simulink model "AmpelkreuzungV5_99"  (R2024b)
settings: Solver=FixedStepAuto  StartTime=0.0  StopTime=5000  FixedStep=1  RelTol=1e-3
model workspace (MATLAB code in the model file):
  | function [autos_l1, autos_rg1, autos_2l, autos_2rg, autos_3l, autos_3rg, autos_4, fehler] = generateCars(Auslastung)
  |     if (auslastung == 1)
  |         autos_l1 = round(randn());
  |         autos_rg1 = round(randn());
  |         autos_2l = round(randn());
  |         autos_2rg = round(randn());
  |         autos_3l = round(randn());
  |         autos_3rg = round(randn());
  |         autos_4 = round(randn());
  |     else
  |         fehler = 1;
  |     end
  | 
  |     if (auslastung == 2)
  |         autos_l1 = round(randn());
  |         autos_rg1 = round(4 + 2 * randn());
  |         autos_2l = round(1 + randn());
  |         autos_2rg = round(4 + 2 * randn());
  |         autos_3l = round(randn());
  |         autos_3rg = round(2 + randn());
  |         autos_4 = round(1 + randn());
  |     else
  |         fehler = 1;
  |     end
  | 
  |     if (auslastung == 3)
  |         autos_l1 = round(1.5 + randn());
  |         autos_rg1 = round(7 + 2 * randn());
  |         autos_2l = round(2 + randn());
  |         autos_2rg = round(7 + 2 * randn());
  |         autos_3l = round(2 * randn());
  |         autos_3rg = round(3 + randn());
  |         autos_4 = round(2 + randn());
  |     else
  |         fehler = 1;
  |     end
  | 
  |     if (auslastung == 4)
  |         autos_l1 = round(2.5 + randn());
  |         autos_rg1 = round(13 + 3 * randn());
  |         autos_2l = round(5 + randn());
  |         autos_2rg = round(13 + 3 * randn());
  |         autos_3l = round(2 + randn());
  |         autos_3rg = round(2 + randn());
  |         autos_4 = round(5 + randn());
  |     else
  |         fehler = 1;
  |     end
  | end
(part 2 of 3)

== stateflow chart AmpelkreuzungV5_99/Chart ==
  state Start
    entry:
    clear all;
    rot1_l = 1;
    gelb1_l = 0;
    gruen1_l = 0;
    rot1_rg = 1;
    gelb1_rg = 0;
    gruen1_rg = 0;
    rot2 = 1;
    gelb2 = 0;
    gruen2 = 0;
    rot3_l = 1;
    gelb3_l = 0;
    gruen3_l = 0;
    rot3_rg = 1;
    gelb3_rg = 0;
    gruen3_rg = 0;
    rot4 = 1;
    gelb4 = 0;
    gruen4 = 0;
    rot5 = 1;
    gruen5 = 0;
    rot6 = 1;
    gruen6 = 0;
    rot7 = 1;
    gruen7 = 0;
    rot8 = 1;
    gruen8 = 0;
    timeCounter = 0;
    timer_spuren = [0 0 0 0 0 0 0];
    gesamtZeit = 0;
    gesamte_autos = 0;
    %alle_autos = [0 0 0 0 0 0 0; 0 0 0 0 0 0 0];
    spur1 = zeros(1,N / 2);
    spur2 = zeros(1,N / 2);
    spur3 = zeros(1,N / 2);
    spur4 = zeros(1,N / 2);
    spur5 = zeros(1,N / 2);
    spur6 = zeros(1,N / 2);
    spur7 = zeros(1,N / 2);
    autos_auf_spur1 = 0;
    autos_auf_spur2 = 0;
    autos_auf_spur3 = 0;
    autos_auf_spur4 = 0;
    autos_auf_spur5 = 0;
    autos_auf_spur6 = 0;
    autos_auf_spur7 = 0;
    counter = [0 0 0 0 0 0 0];
    anz_autos1 = 0;
    anz_autos2 = 0;
    anz_autos3 = 0;
    anz_autos4 = 0;
    anz_autos5 = 0;
    anz_autos6 = 0;
    anz_autos7 = 0;
    wartezeit_spur1_ges = 0;
    wartezeit_spur2_ges = 0;
    wartezeit_spur3_ges = 0;
    wartezeit_spur4_ges = 0;
    wartezeit_spur5_ges = 0;
    wartezeit_spur6_ges = 0;
    wartezeit_spur7_ges = 0;
    krit1 = 0;
    krit2 = 0;
    krit3 = 0;
  state dokumentiere_startzeiten_initialisiere_wartezeiten
    en:
    startzeiten1 = spur1;
    startzeiten2 = spur2;
    startzeiten3 = spur3;
    startzeiten4 = spur4;
    startzeiten5 = spur5;
    startzeiten6 = spur6;
    startzeiten7 = spur7;
    wartezeiten1 = zeros(1, length(startzeiten1));
    wartezeiten2 = zeros(1, length(startzeiten2));
    wartezeiten3 = zeros(1, length(startzeiten3));
    wartezeiten4 = zeros(1, length(startzeiten4));
    wartezeiten5 = zeros(1, length(startzeiten5));
    wartezeiten6 = zeros(1, length(startzeiten6));
    wartezeiten7 = zeros(1, length(startzeiten7));
  state endzeiten_initialisieren
    en:
    endzeiten1 = zeros(1, length(spur1));
    endzeiten2 = zeros(1, length(spur2));
    endzeiten3 = zeros(1, length(spur3));
    endzeiten4 = zeros(1, length(spur4));
    endzeiten5 = zeros(1, length(spur5));
    endzeiten6 = zeros(1, length(spur6));
    endzeiten7 = zeros(1, length(spur7));
  state rg1_ampel2_rotgelb
    entry:
    gelb1_rg = 1;
    gelb2 = 1;
  state l1_rg1_rotgelb
    entry:
    gelb1_l = 1;
    gelb1_rg = 1;
  state rg1_ampel2_gruen
    entry:
    rot1_rg = 0;
    gelb1_rg = 0;
    gruen1_rg = 1;
    rot2 = 0;
    gelb2 = 0;
    gruen2 = 1;
    rot7 = 0;
    gruen7 = 1;
    rot8 = 0;
    gruen8 = 1;
  state rg1_ampel2_rotgelb4
    entry:
    gelb1_rg = 1;
    gelb2 = 1;
  state l1_rg1_gruen
    entry:
    rot1_l = 0;
    gelb1_l = 0;
    gruen1_l = 1;
    rot1_rg = 0;
    gelb1_rg = 0;
    gruen1_rg = 1;
    rot7 = 0;
    gruen7 = 1;
  state l1_rg1_rotgelb4
    entry:
    gelb1_l = 1;
    gelb1_rg = 1;
  state rg1_ampel2_rotgelb1
    entry:
    gelb1_rg = 1;
    gelb2 = 1;
  state rg1_ampel2_gruen4
    entry:
    rot1_rg = 0;
    gelb1_rg = 0;
    gruen1_rg = 1;
    rot2 = 0;
    gelb2 = 0;
    gruen2 = 1;
    rot7 = 0;
    gruen7 = 1;
    rot8 = 0;
    gruen8 = 1;
  state l1_rg1_rotgelb1
    entry:
    gelb1_l = 1;
    gelb1_rg = 1;
  state l1_gelb
    entry:
    gelb1_l = 1;
    gruen1_l = 0;
  state rg1_ampel2_gruen1
    entry:
    rot1_rg = 0;
    gelb1_rg = 0;
    gruen1_rg = 1;
    rot2 = 0;
    gelb2 = 0;
    gruen2 = 1;
    rot7 = 0;
    gruen7 = 1;
    rot8 = 0;
    gruen8 = 1;
  state l1_rg1_gruen4
    entry:
    rot1_l = 0;
    gelb1_l = 0;
    gruen1_l = 1;
    rot1_rg = 0;
    gelb1_rg = 0;
    gruen1_rg = 1;
    rot7 = 0;
    gruen7 = 1;
  state l1_rg1_gruen1
    entry:
    rot1_l = 0;
    gelb1_l = 0;
    gruen1_l = 1;
    rot1_rg = 0;
    gelb1_rg = 0;
    gruen1_rg = 1;
    rot7 = 0;
    gruen7 = 1;
  state rg1_ampel2_rotgelb3
    entry:
    gelb1_rg = 1;
    gelb2 = 1;
  state l1_rot
    entry:
    rot1_l = 1;
    gelb1_l = 0;
  state l1_rg1_rotgelb3
    entry:
    gelb1_l = 1;
    gelb1_rg = 1;
  state Fuss7_rot1
    entry:
    rot7 = 1;
    gruen7 = 0;
  state l1_gelb4
    entry:
    gelb1_l = 1;
    gruen1_l = 0;
  state rg1_ampel2_gruen3
    entry:
    rot1_rg = 0;
    gelb1_rg = 0;
    gruen1_rg = 1;
    rot2 = 0;
    gelb2 = 0;
    gruen2 = 1;
    rot7 = 0;
    gruen7 = 1;
    rot8 = 0;
    gruen8 = 1;
  state l1_gelb1
    entry:
    gelb1_l = 1;
    gruen1_l = 0;
  state l1_rg1_gruen3
    entry:
    rot1_l = 0;
    gelb1_l = 0;
    gruen1_l = 1;
    rot1_rg = 0;
    gelb1_rg = 0;
    gruen1_rg = 1;
    rot7 = 0;
    gruen7 = 1;
  state l1_rot1
    entry:
    rot1_l = 1;
    gelb1_l = 0;
  state l1_rot9
    entry:
    rot1_l = 1;
    gelb1_l = 0;
  state rg1_gelb1
    entry:
    gelb1_rg = 1;
    gruen1_rg = 0;
  state Fuss7_rot8
    entry:
    rot7 = 1;
    gruen7 = 0;
  state l1_rot2
    entry:
    rot1_l = 1;
    gelb1_l = 0;
  state ampel2_rotgelb
    entry:
    gelb2 = 1;
  state Fuss7_rot2
    entry:
    rot7 = 1;
    gruen7 = 0;
  state ampel2_fuss8_gruen
    rot2 = 0;
    gelb2 = 0;
    gruen2 = 1;
    rot8 = 0;
    gruen8 = 1;
  state l1_gelb3
    entry:
    gelb1_l = 1;
    gruen1_l = 0;
  state rg1_rot1
    entry:
    gelb1_rg = 0;
    rot1_rg = 1;
  state l1_rot8
    entry:
    rot1_l = 1;
    gelb1_l = 0;
  state rg1_gelb9
    entry:
    gelb1_rg = 1;
    gruen1_rg = 0;
  state l1_rot3
    entry:
    rot1_l = 1;
    gelb1_l = 0;
  state ampel2_rotgelb4
    entry:
    gelb2 = 1;
  state rg1_gelb2
    entry:
    gelb1_rg = 1;
    gruen1_rg = 0;
  state l1_rot6
    entry:
    rot1_l = 1;
    gelb1_l = 0;
  state Fuss7_rot6
    entry:
    rot7 = 1;
    gruen7 = 0;
  state ampel2_rotgelb1
    entry:
    gelb2 = 1;
  state ampel2_fuss8_gruen4
    rot2 = 0;
    gelb2 = 0;
    gruen2 = 1;
    rot8 = 0;
    gruen8 = 1;
  state rg1_rot23
    entry:
    gelb1_rg = 0;
    rot1_rg = 1;
  state ampel2_fuss8_gruen1
    rot2 = 0;
    gelb2 = 0;
    gruen2 = 1;
    rot8 = 0;
    gruen8 = 1;
  state Fuss7_rot
    entry:
    rot7 = 1;
    gruen7 = 0;
  state rg1_rot6
    entry:
    gelb1_rg = 0;
    rot1_rg = 1;
  state l1_rot7
    entry:
    rot1_l = 1;
    gelb1_l = 0;
  state rg1_gelb7
    entry:
    gelb1_rg = 1;
    gruen1_rg = 0;
  state rg1_gelb
    entry:
    gelb1_rg = 1;
    gruen1_rg = 0;
  state fuss7_rot
    entry:
    rot7 = 1;
    gruen7 = 0;
  state Fuss7_rot7
    entry:
    rot7 = 1;
    gruen7 = 0;
  state rg1_rot20
    entry:
    gelb1_rg = 0;
    rot1_rg = 1;
  state rg1_rot
    entry:
    gelb1_rg = 0;
    rot1_rg = 1;
  state Fuss7_rot3
    entry:
    rot7 = 1;
    gruen7 = 0;
  state rg1_rot5
    entry:
    gelb1_rg = 0;
    rot1_rg = 1;
  state rg1_gelb8
    entry:
    gelb1_rg = 1;
    gruen1_rg = 0;
  state ampel2_rotgelb3
    entry:
    gelb2 = 1;
  state rg1_gelb3
    entry:
    gelb1_rg = 1;
    gruen1_rg = 0;
  state ampel2_fuss8_gruen3
    rot2 = 0;
    gelb2 = 0;
    gruen2 = 1;
    rot8 = 0;
    gruen8 = 1;
  state rg1_rot26
    entry:
    gelb1_rg = 0;
    rot1_rg = 1;
  state rg1_rot7
    entry:
    gelb1_rg = 0;
    rot1_rg = 1;
  state fuss8_rot7
    entry:
    rot8 = 1;
    gruen8 = 0;
  state rg1_rot4
    entry:
    gelb1_rg = 0;
    rot1_rg = 1;
  state rg1_gelb6
    entry:
    gelb1_rg = 1;
    gruen1_rg = 0;
  state rg1_rot11
    entry:
    gelb1_rg = 0;
    rot1_rg = 1;
  state rg1_rot17
    entry:
    gelb1_rg = 0;
    rot1_rg = 1;
  state rg1_rot22
    entry:
    gelb1_rg = 0;
    rot1_rg = 1;
  state fuss8_rot11
    entry:
    rot8 = 1;
    gruen8 = 0;
  state rg1_rot9
    entry:
    gelb1_rg = 0;
    rot1_rg = 1;
  state fuss8_rot13
    entry:
    rot8 = 1;
    gruen8 = 0;
  state rg1_rot24
    entry:
    gelb1_rg = 0;
    rot1_rg = 1
  state fuss8_rot14
    entry:
    rot8 = 1;
    gruen8 = 0;
  state rg1_rot25
    entry:
    gelb1_rg = 0;
    rot1_rg = 1
  state rg1_rot21
    entry:
    gelb1_rg = 0;
    rot1_rg = 1;
  state fuss8_rot5
    entry:
    rot8 = 1;
    gruen8 = 0;
  state fuss8_rot4
    entry:
    rot8 = 1;
    gruen8 = 0;
  state ampel2_gelb12
    entry:
    gelb2 = 1;
    gruen2 = 0;
  state ampel2_gelb13
    entry:
    gelb2 = 1;
    gruen2 = 0;
  state ampel2_gelb5
    entry:
    gelb2 = 1;
    gruen2 = 0;
  state ampel2_gelb4
    entry:
    gelb2 = 1;
    gruen2 = 0;
  state rg1_rot19
    entry:
    gelb1_rg = 0;
    rot1_rg = 1
  state ampel2_gelb8
    entry:
    gelb2 = 1;
    gruen2 = 0;
  state rg1_rot3
    entry:
    gelb1_rg = 0;
    rot1_rg = 1
  state rg1_rot18
    entry:
    gelb1_rg = 0;
    rot1_rg = 1
  state ampel2_gelb11
    entry:
    gelb2 = 1;
    gruen2 = 0;
  state rg1_rot2
    entry:
    gelb1_rg = 0;
    rot1_rg = 1
  state fuss8_rot10
    entry:
    rot8 = 1;
    gruen8 = 0;
  state fuss8_rot12
    entry:
    rot8 = 1;
    gruen8 = 0;
  state ampel2_rot24
    rot2 = 1;
    gelb2 = 0;
  state fuss8_rot1
    entry:
    rot8 = 1;
    gruen8 = 0;
  state ampel2_rot11
    rot2 = 1;
    gelb2 = 0;
  state fuss8_rot
    entry:
    rot8 = 1;
    gruen8 = 0;
  state ampel2_gelb9
    entry:
    gelb2 = 1;
    gruen2 = 0;
  state ampel2_gelb10
    entry:
    gelb2 = 1;
    gruen2 = 0;
  state ampel2_gelb1
    entry:
    gelb2 = 1;
    gruen2 = 0;
  state rg1_rot8
    entry:
    gelb1_rg = 0;
    rot1_rg = 1
  state ampel2_gelb
    entry:
    gelb2 = 1;
    gruen2 = 0;
  state rg1_rot10
    entry:
    gelb1_rg = 0;
    rot1_rg = 1
  state ampel2_rot25
    rot2 = 1;
    gelb2 = 0;
  state ampel2_rot9
    rot2 = 1;
    gelb2 = 0;
  state fuss8_rot3
    entry:
    rot8 = 1;
    gruen8 = 0;
  state ampel2_rot19
    rot2 = 1;
    gelb2 = 0;
  state fuss8_rot2
    entry:
    rot8 = 1;
    gruen8 = 0;
  state ampel2_rot17
    rot2 = 1;
    gelb2 = 0;
  state ampel2_rot
    rot2 = 1;
    gelb2 = 0;
  state ampel2_gelb3
    entry:
    gelb2 = 1;
    gruen2 = 0;
  state ampel2_gelb2
    entry:
    gelb2 = 1;
    gruen2 = 0;
  state ampel2_rot21
    rot2 = 1;
    gelb2 = 0;
  state ampel2_rot20
    rot2 = 1;
    gelb2 = 0;
  state ampel2_rot1
    rot2 = 1;
    gelb2 = 0;
  state ampel2_rot5
    rot2 = 1;
    gelb2 = 0;
  state ampel2_rot26
    rot2 = 1;
    gelb2 = 0;
  state ampel2_rot10
    rot2 = 1;
    gelb2 = 0;
  state ampel2_rot27
    rot2 = 1;
    gelb2 = 0;
  state ampel2_rot8
    rot2 = 1;
    gelb2 = 0;
  state rg3_rotgelb13
    entry:
    gelb3_rg = 1;
  state rg3_rotgelb4
    entry:
    gelb3_rg = 1;
  state ampel2_rot6
    rot2 = 1;
    gelb2 = 0;
  state rg3_rotgelb14
    entry:
    gelb3_rg = 1;
  state rg3_rotgelb5
    entry:
    gelb3_rg = 1;
  state ampel2_rot16
    rot2 = 1;
    gelb2 = 0;
  state ampel2_rot22
    rot2 = 1;
    gelb2 = 0;
  state ampel2_rot18
    rot2 = 1;
    gelb2 = 0;
  state ampel2_rot2
    rot2 = 1;
    gelb2 = 0;
  state ampel2_rot23
    rot2 = 1;
    gelb2 = 0;
  state ampel2_rot3
    rot2 = 1;
    gelb2 = 0;
  state rg3_rotgelb10
    entry:
    gelb3_rg = 1;
  state rg3_rotgelb11
    entry:
    gelb3_rg = 1;
  state rg3_rotgelb12
    entry:
    gelb3_rg = 1;
  state rg3_rotgelb
    entry:
    gelb3_rg = 1;
  state rg3_rotgelb9
    entry:
    gelb3_rg = 1;
  state rg3_rotgelb1
    entry:
    gelb3_rg = 1;
  state ampel2_rot7
    rot2 = 1;
    gelb2 = 0;
  state ampel2_rot4
    rot2 = 1;
    gelb2 = 0;
  state rg3_rotgelb2
    entry:
    gelb3_rg = 1;
  state l3_rotgelb_rg3_fuss6_gruen
    entry:
    gelb3_l = 1;
    rot3_rg = 0;
    gelb3_rg = 0;
    gruen3_rg = 1;
    rot6 = 0;
    gruen6 = 1;
  state rg3_fuss6_gruen
    entry:
    rot3_rg = 0;
    gelb3_rg = 0;
    gruen3_rg = 1;
    rot6 = 0;
    gruen6 = 1;
  state rg3_rotgelb3
    entry:
    gelb3_rg = 1;
  state rg3_rotgelb6
    entry:
    gelb3_rg = 1;
  state ampel4_rotgelb
    entry:
    gelb4 = 1;
  state l3_rotgelb_rg3_fuss6_gruen4
    entry:
    gelb3_l = 1;
    rot3_rg = 0;
    gelb3_rg = 0;
    gruen3_rg = 1;
    rot6 = 0;
    gruen6 = 1;
  state rg3_fuss6_gruen4
    entry:
    rot3_rg = 0;
    gelb3_rg = 0;
    gruen3_rg = 1;
    rot6 = 0;
    gruen6 = 1;
  state l3_gruen
    entry:
    rot3_l = 0;
    gelb3_l = 0;
    gruen3_l = 1;
  state l3_rotgelb_rg3_fuss6_gruen1
    entry:
    gelb3_l = 1;
    rot3_rg = 0;
    gelb3_rg = 0;
    gruen3_rg = 1;
    rot6 = 0;
    gruen6 = 1;
  state rg3_fuss6_gruen1
    entry:
    rot3_rg = 0;
    gelb3_rg = 0;
    gruen3_rg = 1;
    rot6 = 0;
    gruen6 = 1;
  state ampel4_rotgelb4
    entry:
    gelb4 = 1;
  state l3_gruen4
    entry:
    rot3_l = 0;
    gelb3_l = 0;
    gruen3_l = 1;
  state l3_gelb
    entry:
    gelb3_l = 1;
    gruen3_l = 0;
  state ampel4_rotgelb1
    entry:
    gelb4 = 1;
  state l3_gruen1
    entry:
    rot3_l = 0;
    gelb3_l = 0;
    gruen3_l = 1;
  state ampel4_fuss5_gruen
    entry:
    rot4 = 0;
    gelb4 = 0;
    gruen4 = 1;
    rot5 = 0;
    gruen5 = 1;
  state l3_rotgelb_rg3_fuss6_gruen3
    entry:
    gelb3_l = 1;
    rot3_rg = 0;
    gelb3_rg = 0;
    gruen3_rg = 1;
    rot6 = 0;
    gruen6 = 1;
  state rg3_fuss6_gruen3
    entry:
    rot3_rg = 0;
    gelb3_rg = 0;
    gruen3_rg = 1;
    rot6 = 0;
    gruen6 = 1;
  state l3_fuss6_rot
    entry:
    rot3_l = 1;
    gelb3_l = 0;
    rot6 = 1;
    gruen6 = 0;
  state l3_gelb_fuss6_rot
    entry:
    gelb3_l = 1;
    gruen3_l = 0;
  state ampel4_rotgelb3
    entry:
    gelb4 = 1;
  state ampel4_fuss5_gruen8
    entry:
    rot4 = 0;
    gelb4 = 0;
    gruen4 = 1;
    rot5 = 0;
    gruen5 = 1;
  state l3_gelb1
    entry:
    gelb3_l = 1;
    gruen3_l = 0;
  state l3_gruen3
    entry:
    rot3_l = 0;
    gelb3_l = 0;
    gruen3_l = 1;
  state fuss6_rot6
    entry:
    rot6 = 1;
    gruen6 = 0;
  state ampel4_fuss5_gruen2
    entry:
    rot4 = 0;
    gelb4 = 0;
    gruen4 = 1;
    rot5 = 0;
    gruen5 = 1;
  state l3_fuss6_rot3
    entry:
    rot3_l = 1;
    gelb3_l = 0;
    rot6 = 1;
    gruen6 = 0;
  state l3_rot1
    entry:
    rot3_l = 1;
    gelb3_l = 0;
  state l3_gelb2
    entry:
    gelb3_l = 1;
    gruen3_l = 0;
  state l3_fuss6_rot1
    entry:
    rot3_l = 1;
    gelb3_l = 0;
    rot6 = 1;
    gruen6 = 0;
  state ampel4_fuss5_gruen6
    entry:
    rot4 = 0;
    gelb4 = 0;
    gruen4 = 1;
    rot5 = 0;
    gruen5 = 1;
  state fuss6_rot
    entry:
    rot6 = 1;
    gruen6 = 0;
  state fuss6_rot4
    entry:
    rot6 = 1;
    gruen6 = 0;
  state rg3_gelb1
    entry:
    gelb3_rg = 1;
    gruen3_rg = 0;
  state rg3_gelb
    entry:
    gelb3_rg = 1;
    gruen3_rg = 0;
  state l3_rot_rg3_gelb
    entry:
    rot3_l = 1;
    gelb3_l = 0;
    gelb3_rg = 1;
    gruen3_rg = 0;
  state l3_rot
    entry:
    rot3_l = 1;
    gelb3_l = 0;
  state fuss6_rot7
    entry:
    rot6 = 1;
    gruen6 = 0;
  state l3_fuss6_rot2
    entry:
    rot3_l = 1;
    gelb3_l = 0;
    rot6 = 1;
    gruen6 = 0;
  state fuss6_rot1
    entry:
    rot6 = 1;
    gruen6 = 0;
  state rg3_gelb8
    entry:
    gelb3_rg = 1;
    gruen3_rg = 0;
  state rg3_gelb7
    entry:
    gelb3_rg = 1;
    gruen3_rg = 0;
  state rg3_rot_ampel4_rotgelb
    entry:
    rot3_rg = 1;
    gelb3_rg = 0;
    gelb4 = 1;
  state rg3_gelb2
    entry:
    gelb3_rg = 1;
    gruen3_rg = 0;
  state rg3_gelb3
    entry:
    gelb3_rg = 1;
    gruen3_rg = 0;
  state rg3_fuss5_rot
    entry:
    rot3_rg = 1;
    gelb3_rg = 0;
    rot5 = 1;
    gruen5 = 0;
  state fuss6_rot5
    entry:
    rot6 = 1;
    gruen6 = 0;
  state rg3_rot_ampel4_rotgelb8
    entry:
    rot3_rg = 1;
    gelb3_rg = 0;
    gelb4 = 1;
  state l3_rot_rg3_gelb1
    entry:
    rot3_l = 1;
    gelb3_l = 0;
    gelb3_rg = 1;
    gruen3_rg = 0;
  state rg3_gelb6
    entry:
    gelb3_rg = 1;
    gruen3_rg = 0;
  state rg3_rot_ampel4_rotgelb2
    entry:
    rot3_rg = 1;
    gelb3_rg = 0;
    gelb4 = 1;
  state rg3_fuss5_rot8
    entry:
    rot3_rg = 1;
    gelb3_rg = 0;
    rot5 = 1;
    gruen5 = 0;
  state rg3_rot_ampel4_rotgelb1
    entry:
    rot3_rg = 1;
    gelb3_rg = 0;
    gelb4 = 1;
  state rg3_fuss5_rot2
    entry:
    rot3_rg = 1;
    gelb3_rg = 0;
    rot5 = 1;
    gruen5 = 0;
  state rg3_rot_ampel4_rotgelb6
    entry:
    rot3_rg = 1;
    gelb3_rg = 0;
    gelb4 = 1;
  state ampel4_fuss5_gruen1
    entry:
    rot4 = 0;
    gelb4 = 0;
    gruen4 = 1;
    rot5 = 0;
    gruen5 = 1;
  state rg3_rot_ampel4_rotgelb9
    entry:
    rot3_rg = 1;
    gelb3_rg = 0;
    gelb4 = 1;
  state rg3_fuss5_rot6
    entry:
    rot3_rg = 1;
    gelb3_rg = 0;
    rot5 = 1;
    gruen5 = 0;
  state rg3_rot_ampel4_rotgelb3
    entry:
    rot3_rg = 1;
    gelb3_rg = 0;
    gelb4 = 1;
  state ampel4_fuss5_gruen9
    entry:
    rot4 = 0;
    gelb4 = 0;
    gruen4 = 1;
    rot5 = 0;
    gruen5 = 1;
  state fuss5_rot
    entry:
    rot5 = 1;
    gruen5 = 0;
  state ampel4_fuss5_gruen3
    entry:
    rot4 = 0;
    gelb4 = 0;
    gruen4 = 1;
    rot5 = 0;
    gruen5 = 1;
  state rg3_rot_ampel4_rotgelb7
    entry:
    rot3_rg = 1;
    gelb3_rg = 0;
    gelb4 = 1;
  state rg3_fuss5_rot1
    entry:
    rot3_rg = 1;
    gelb3_rg = 0;
    rot5 = 1;
    gruen5 = 0;
  state fuss5_rot4
    entry:
    rot5 = 1;
    gruen5 = 0;
  state ampel4_fuss5_gruen7
    entry:
    rot4 = 0;
    gelb4 = 0;
    gruen4 = 1;
    rot5 = 0;
    gruen5 = 1;
  state fuss5_rot1
    entry:
    rot5 = 1;
    gruen5 = 0;
  state rg3_fuss5_rot9
    entry:
    rot3_rg = 1;
    gelb3_rg = 0;
    rot5 = 1;
    gruen5 = 0;
  state rg3_fuss5_rot3
    entry:
    rot3_rg = 1;
    gelb3_rg = 0;
    rot5 = 1;
    gruen5 = 0;
  state fuss5_rot3
    entry:
    rot5 = 1;
    gruen5 = 0;
  state ampel4_gelb
    entry:
    gelb4 = 1;
    gruen4 = 0;
  state rg3_fuss5_rot7
    entry:
    rot3_rg = 1;
    gelb3_rg = 0;
    rot5 = 1;
    gruen5 = 0;
  state ampel4_rot
    entry:
    rot4 = 1;
    gelb4 = 0;
  state ampel4_gelb4
    entry:
    gelb4 = 1;
    gruen4 = 0;
  state ampel4_rot2
    entry:
    rot4 = 1;
    gelb4 = 0;
  state ampel4_gelb1
    entry:
    gelb4 = 1;
    gruen4 = 0;
  state ampel4_rot9
    entry:
    rot4 = 1;
    gelb4 = 0;
  state ampel4_rot3
    entry:
    rot4 = 1;
    gelb4 = 0;
  state ampel4_rot10
    entry:
    rot4 = 1;
    gelb4 = 0;
  state ampel4_gelb3
    entry:
    gelb4 = 1;
    gruen4 = 0;
  state ampel4_rot4
    entry:
    rot4 = 1;
    gelb4 = 0;
  state ampel4_rot7
    entry:
    rot4 = 1;
    gelb4 = 0;
  state ampel4_rot8
    entry:
    rot4 = 1;
    gelb4 = 0;
  (default) -> Start
  Start -> (junction 796) : {zeit_abstand = zeit_abstand_aus_auslastung(auslastung);}
  (junction 796) -> (junction 748) : {alle_autos_neu  = generiere_autos_neu(N, zeit_abstand, auslastung);}
  (junction 748) -> dokumentiere_startzeiten_initialisiere_wartezeiten : {[spur1, spur2, spur3, spur4, spur5, spur6, spur7] = spuren_aus_autos(alle_autos_neu, N);}
  dokumentiere_startzeiten_initialisiere_wartezeiten -> endzeiten_initialisieren
  endzeiten_initialisieren -> (junction 248)
  (junction 181) -> (junction 248) : {timeCounter = resetTimer()}
  (junction 248) -> (junction 1426) [order 1] : [auslastung == 5]
  (junction 248) -> (junction 1428) [order 2]
  (junction 179) -> (junction 181)
  (junction 1426) -> (junction 1092) : {alte_counter = counter;}
  (junction 1428) -> (junction 1430) [order 1] : [auslastung == 4]
  (junction 1428) -> (junction 1840) [order 2]
  (junction 1430) -> (junction 1670) : {alte_counter = counter;}
  (junction 1840) -> (junction 1843) [order 1] : [auslastung == 3]
  (junction 1840) -> (junction 3331) [order 2]
  (junction 1843) -> (junction 3396) : {alte_counter = counter;}
  (junction 3331) -> (junction 3333) : [auslastung == 1 || auslastung == 2]
  (junction 3333) -> (junction 3239) : {alte_counter = counter;}
  (junction 1092) -> (junction 1075) : after(1,sec)
      | {timeCounter = refresher(timeCounter, 1);}
  (junction 1075) -> (junction 1077) : {timer_spuren = countOnwards(timer_spuren,1,[1 1 1 1 1 1 1]);}
      |
      | %Linksabbieger1
  (junction 1077) -> (junction 1076) : {[autos_auf_spur1, spur1] = autos_auf_spur_generieren(spur1, gesamtZeit + timeCounter + 2, autos_auf_spur1);}
  (junction 3396) -> (junction 3418) : after(1,sec)
      | {timeCounter = refresher(timeCounter, 1);}
  (junction 1076) -> (junction 1081) : {autos_spur1_flag = false;}
  (junction 3418) -> (junction 3423) : {timer_spuren = countOnwards(timer_spuren,1,[1 1 1 1 1 1 1]);}
      |
      | %Linksabbieger1
  (junction 1670) -> (junction 1696) : after(1,sec)
      | {timeCounter = refresher(timeCounter, 1);}
  (junction 1081) -> (junction 1085) [order 1] : [autos_auf_spur1 == 0]
  (junction 1696) -> (junction 1673) : {timer_spuren = countOnwards(timer_spuren,1,[1 1 1 1 1 1 1]);}
      |
      | %Linksabbieger1
  (junction 3423) -> (junction 3398) : {[autos_auf_spur1, spur1] = autos_auf_spur_generieren(spur1, gesamtZeit + timeCounter + 2, autos_auf_spur1);}
  (junction 1081) -> (junction 1084) [order 2]
  (junction 1085) -> rg1_ampel2_rotgelb
  (junction 1084) -> (junction 1074) [order 1] : [autos_auf_spur1 > 0]
  (junction 1084) -> (junction 1111) [order 2]
  (junction 1074) -> l1_rg1_rotgelb : {autos_spur1_flag = true;}
  rg1_ampel2_rotgelb -> (junction 1097) : after(1,sec)
      | {timeCounter = refresher(timeCounter, 1);}
  (junction 1673) -> (junction 1668) : {[autos_auf_spur1, spur1] = autos_auf_spur_generieren(spur1, gesamtZeit + timeCounter + 2, autos_auf_spur1);}
  (junction 1097) -> rg1_ampel2_gruen : {timer_spuren = countOnwards(timer_spuren,1,[1 1 1 1 1 1 1]);}
  (junction 3398) -> (junction 3386) : {autos_spur1_flag = false;}
  l1_rg1_rotgelb -> (junction 1082) : after(1,sec)
      | {timeCounter = refresher(timeCounter, 1);}
  (junction 1082) -> l1_rg1_gruen : {timer_spuren = countOnwards(timer_spuren,1,[1 1 1 1 1 1 1]);}
  (junction 3239) -> (junction 3238) : after(1,sec)
      | {timeCounter = refresher(timeCounter, 1);}
  (junction 1668) -> (junction 1687) : {autos_spur1_flag = false;}
  (junction 3386) -> (junction 3402) [order 1] : [autos_auf_spur1 == 0]
  (junction 3402) -> rg1_ampel2_rotgelb4
  (junction 3386) -> (junction 3387) [order 2]
  (junction 3238) -> (junction 3241) : {timer_spuren = countOnwards(timer_spuren,1,[1 1 1 1 1 1 1]);}
      |
      | %Linksabbieger1
  (junction 3387) -> (junction 3395) [order 1] : [autos_auf_spur1 > 0]
  (junction 3387) -> (junction 3436) [order 2]
  (junction 3395) -> l1_rg1_rotgelb4 : {autos_spur1_flag = true;}
  rg1_ampel2_rotgelb4 -> (junction 3400) : after(1,sec)
      | {timeCounter = refresher(timeCounter, 1);}
  rg1_ampel2_gruen -> (junction 1080) : {[autos_auf_spur2, spur2] = autos_auf_spur_generieren(spur2, gesamtZeit + timeCounter, autos_auf_spur2);}
  (junction 1687) -> (junction 1688) [order 1] : [autos_auf_spur1 == 0]
  (junction 1687) -> (junction 1690) [order 2]
  (junction 1688) -> rg1_ampel2_rotgelb1
  (junction 3241) -> (junction 3240) : {[autos_auf_spur1, spur1] = autos_auf_spur_generieren(spur1, gesamtZeit + timeCounter + 2, autos_auf_spur1);}
  (junction 1080) -> (junction 1098) : {[autos_auf_spur3, spur3] = autos_auf_spur_generieren(spur3, gesamtZeit + timeCounter, autos_auf_spur3);}
  (junction 3400) -> rg1_ampel2_gruen4 : {timer_spuren = countOnwards(timer_spuren,1,[1 1 1 1 1 1 1]);}
  l1_rg1_gruen -> (junction 1083) : {[autos_auf_spur1, spur1] = autos_auf_spur_generieren(spur1, gesamtZeit + timeCounter, autos_auf_spur1);}
  (junction 1690) -> (junction 1697) [order 1] : [autos_auf_spur1 > 0]
  (junction 1690) -> (junction 1741) [order 2]
  (junction 1697) -> l1_rg1_rotgelb1 : {autos_spur1_flag = true;}
  l1_rg1_rotgelb4 -> (junction 3404) : after(1,sec)
      | {timeCounter = refresher(timeCounter, 1);}
  rg1_ampel2_rotgelb1 -> (junction 1698) : after(1,sec)
      | {timeCounter = refresher(timeCounter, 1);}
  (junction 1083) -> (junction 1078) : {[autos_auf_spur2, spur2] = autos_auf_spur_generieren(spur2, gesamtZeit + timeCounter, autos_auf_spur2);}
  (junction 1098) -> (junction 1086) : {[autos_auf_spur4, spur4] = autos_auf_spur_generieren(spur4, gesamtZeit + timeCounter, autos_auf_spur4);}
  (junction 3404) -> l1_rg1_gruen4 : {timer_spuren = countOnwards(timer_spuren,1,[1 1 1 1 1 1 1]);}
  (junction 1078) -> (junction 1073) : after(8,sec)
      | {timeCounter = refresher(timeCounter, 8);}
  (junction 1698) -> rg1_ampel2_gruen1 : {timer_spuren = countOnwards(timer_spuren,1,[1 1 1 1 1 1 1]);}
  l1_rg1_rotgelb1 -> (junction 1715) : after(1,sec)
      | {timeCounter = refresher(timeCounter, 1);}
  (junction 3240) -> (junction 3243) : {autos_spur1_flag = false;}
  (junction 1073) -> l1_gelb : {timer_spuren = countOnwards(timer_spuren,8,[0 0 1 1 1 1 1]);}
  (junction 1086) -> (junction 1087) : after(45,sec)
      | {timeCounter = refresher(timeCounter, 45);}
  (junction 1715) -> l1_rg1_gruen1 : {timer_spuren = countOnwards(timer_spuren,1,[1 1 1 1 1 1 1]);}
  l1_gelb -> (junction 1093) : after(3,sec)
      | {timeCounter = refresher(timeCounter, 3);}
  (junction 1087) -> Fuss7_rot1 : {timer_spuren = countOnwards(timer_spuren,45,[1 0 0 0 1 1 1]);}
  rg1_ampel2_gruen4 -> (junction 3408) : {[autos_auf_spur2, spur2] = autos_auf_spur_generieren(spur2, gesamtZeit + timeCounter, autos_auf_spur2);}
  (junction 1093) -> (junction 1079) : {[autos_auf_spur1, spur1] = autos_auf_spur_generieren(spur1, gesamtZeit + timeCounter, autos_auf_spur1);}
  (junction 3243) -> (junction 3249) [order 1] : [autos_auf_spur1 == 0]
  (junction 3243) -> (junction 3244) [order 2]
  (junction 3249) -> rg1_ampel2_rotgelb3
  (junction 3408) -> (junction 3441) : {[autos_auf_spur3, spur3] = autos_auf_spur_generieren(spur3, gesamtZeit + timeCounter, autos_auf_spur3);}
  (junction 1079) -> l1_rot : {timer_spuren = countOnwards(timer_spuren,3,[0 0 1 1 1 1 1]);}
  l1_rg1_gruen4 -> (junction 3414) : {[autos_auf_spur1, spur1] = autos_auf_spur_generieren(spur1, gesamtZeit + timeCounter, autos_auf_spur1);}
  (junction 3244) -> (junction 3245) [order 1] : [autos_auf_spur1 > 0]
  rg1_ampel2_gruen1 -> (junction 1704) : {[autos_auf_spur2, spur2] = autos_auf_spur_generieren(spur2, gesamtZeit + timeCounter, autos_auf_spur2);}
  (junction 3244) -> (junction 3120) [order 2]
  (junction 3245) -> l1_rg1_rotgelb3 : {autos_spur1_flag = true;}
  rg1_ampel2_rotgelb3 -> (junction 3246) : after(1,sec)
      | {timeCounter = refresher(timeCounter, 1);}
  (junction 3414) -> (junction 3438) : {[autos_auf_spur2, spur2] = autos_auf_spur_generieren(spur2, gesamtZeit + timeCounter, autos_auf_spur2);}
  (junction 3441) -> (junction 3454) : {[autos_auf_spur4, spur4] = autos_auf_spur_generieren(spur4, gesamtZeit + timeCounter, autos_auf_spur4);}
  l1_rot -> (junction 1095) : {[anz_autos1, autos_auf_spur1, counter(1), endzeiten1] = generiere_gruenphase(1, 11, autos_auf_spur1, counter(1),  (gesamtZeit + timeCounter - 11), endzeiten1, startzeiten1, auslastung, autos_spur1_flag);}
  (junction 1704) -> (junction 1722) : {[autos_auf_spur3, spur3] = autos_auf_spur_generieren(spur3, gesamtZeit + timeCounter, autos_auf_spur3);}
  (junction 3438) -> (junction 3442) : after(8,sec)
      | {timeCounter = refresher(timeCounter, 8);}
  l1_rg1_gruen1 -> (junction 1720) : {[autos_auf_spur1, spur1] = autos_auf_spur_generieren(spur1, gesamtZeit + timeCounter, autos_auf_spur1);}
  (junction 3246) -> rg1_ampel2_gruen3 : {timer_spuren = countOnwards(timer_spuren,1,[1 1 1 1 1 1 1]);}
  (junction 1095) -> (junction 1096) : {wartezeiten1 = berechne_wartezeiten(startzeiten1, endzeiten1, alte_counter(1), counter(1), wartezeiten1);}
  (junction 3454) -> (junction 3426) : after(20,sec)
      | {timeCounter = refresher(timeCounter, 20);}
  l1_rg1_rotgelb3 -> (junction 3247) : after(1,sec)
      | {timeCounter = refresher(timeCounter, 1);}
  (junction 3442) -> l1_gelb4 : {timer_spuren = countOnwards(timer_spuren,8,[0 0 1 1 1 1 1]);}
  (junction 1720) -> (junction 1711) : {[autos_auf_spur2, spur2] = autos_auf_spur_generieren(spur2, gesamtZeit + timeCounter, autos_auf_spur2);}
  (junction 1722) -> (junction 1712) : {[autos_auf_spur4, spur4] = autos_auf_spur_generieren(spur4, gesamtZeit + timeCounter, autos_auf_spur4);}
  (junction 1096) -> (junction 1099) : {wartezeit_spur1_ges = gesamt_wartezeit_pro_spur(wartezeiten1, wartezeit_spur1_ges, alte_counter(1), counter(1));}
  Fuss7_rot1 -> (junction 1072) : after(2,sec)
      | {timeCounter = refresher(timeCounter, 2);}
  (junction 3247) -> l1_rg1_gruen3 : {timer_spuren = countOnwards(timer_spuren,1,[1 1 1 1 1 1 1]);}
  (junction 1711) -> (junction 1721) : after(8,sec)
      | {timeCounter = refresher(timeCounter, 8);}
  (junction 3426) -> Fuss7_rot8 : {timer_spuren = countOnwards(timer_spuren,20,[1 0 0 0 1 1 1]);}
  l1_gelb4 -> (junction 3439) : after(3,sec)
      | {timeCounter = refresher(timeCounter, 3);}
  (junction 1099) -> (junction 1090) : {gesamtwartezeit = berechne_gesamtwartezeit(wartezeit_spur1_ges, wartezeit_spur2_ges, wartezeit_spur3_ges, wartezeit_spur4_ges, wartezeit_spur5_ges, wartezeit_spur6_ges, wartezeit_spur7_ges);}
  (junction 1721) -> l1_gelb1 : {timer_spuren = countOnwards(timer_spuren,8,[0 0 1 1 1 1 1]);}
  (junction 1712) -> (junction 1723) : after(35,sec)
      | {timeCounter = refresher(timeCounter, 35);}
  (junction 3439) -> (junction 3452) : {[autos_auf_spur1, spur1] = autos_auf_spur_generieren(spur1, gesamtZeit + timeCounter, autos_auf_spur1);}
  (junction 1072) -> rg1_gelb1 : {timer_spuren = countOnwards(timer_spuren,2,[1 0 0 0 1 1 1]);}
  (junction 1090) -> l1_rot1 : {gesamte_autos = berechne_gesamte_autos(counter(1), counter(2), counter(3), counter(4), counter(5), counter(6), counter(7));}
  l1_gelb1 -> (junction 1724) : after(3,sec)
      | {timeCounter = refresher(timeCounter, 3);}
  (junction 3452) -> l1_rot9 : {timer_spuren = countOnwards(timer_spuren,3,[0 0 1 1 1 1 1]);}
  (junction 1723) -> Fuss7_rot2 : {timer_spuren = countOnwards(timer_spuren,35,[1 0 0 0 1 1 1]);}
  rg1_ampel2_gruen3 -> (junction 3242) : {[autos_auf_spur2, spur2] = autos_auf_spur_generieren(spur2, gesamtZeit + timeCounter, autos_auf_spur2);}
  (junction 1724) -> (junction 1719) : {[autos_auf_spur1, spur1] = autos_auf_spur_generieren(spur1, gesamtZeit + timeCounter, autos_auf_spur1);}
  l1_rot1 -> (junction 1088) : after(3,sec)
      | {timeCounter = refresher(timeCounter, 3);}
  l1_rot9 -> (junction 3437) : {[anz_autos1, autos_auf_spur1, counter(1), endzeiten1] = generiere_gruenphase(1, 11, autos_auf_spur1, counter(1),  (gesamtZeit + timeCounter - 11), endzeiten1, startzeiten1, auslastung, autos_spur1_flag);}
  rg1_gelb1 -> (junction 1089) : after(3,sec)
      | {timeCounter = refresher(timeCounter, 3);}
  (junction 1088) -> ampel2_rotgelb : {timer_spuren = countOnwards(timer_spuren,3,[1 0 1 1 1 1 1]);}
  (junction 3242) -> (junction 3258) : {[autos_auf_spur3, spur3] = autos_auf_spur_generieren(spur3, gesamtZeit + timeCounter, autos_auf_spur3);}
  (junction 1719) -> l1_rot2 : {timer_spuren = countOnwards(timer_spuren,3,[0 0 1 1 1 1 1]);}
  l1_rg1_gruen3 -> (junction 3248) : {[autos_auf_spur1, spur1] = autos_auf_spur_generieren(spur1, gesamtZeit + timeCounter, autos_auf_spur1);}
  (junction 3437) -> (junction 3448) : {wartezeiten1 = berechne_wartezeiten(startzeiten1, endzeiten1, alte_counter(1), counter(1), wartezeiten1);}
  (junction 3248) -> (junction 3259) : {[autos_auf_spur2, spur2] = autos_auf_spur_generieren(spur2, gesamtZeit + timeCounter, autos_auf_spur2);}
  (junction 1089) -> (junction 1094) : {[autos_auf_spur2, spur2] = autos_auf_spur_generieren(spur2, gesamtZeit + timeCounter, autos_auf_spur2);}
  (junction 3258) -> (junction 3264) : {[autos_auf_spur4, spur4] = autos_auf_spur_generieren(spur4, gesamtZeit + timeCounter, autos_auf_spur4);}
  l1_rot2 -> (junction 1725) : {[anz_autos1, autos_auf_spur1, counter(1), endzeiten1] = generiere_gruenphase(1, 11, autos_auf_spur1, counter(1),  (gesamtZeit + timeCounter - 11), endzeiten1, startzeiten1, auslastung, autos_spur1_flag);}
  ampel2_rotgelb -> (junction 1091) : after(1,sec)
      | {timeCounter = refresher(timeCounter, 1);}
  Fuss7_rot8 -> (junction 3453) : after(2,sec)
      | {timeCounter = refresher(timeCounter, 2);}
  (junction 3448) -> (junction 3449) : {wartezeit_spur1_ges = gesamt_wartezeit_pro_spur(wartezeiten1, wartezeit_spur1_ges, alte_counter(1), counter(1));}
  (junction 3259) -> (junction 3265) : after(3,sec)
      | {timeCounter = refresher(timeCounter, 3);}
  (junction 1091) -> ampel2_fuss8_gruen : {timer_spuren = countOnwards(timer_spuren,1,[1 0 1 1 1 1 1]);}
  (junction 1725) -> (junction 1708) : {wartezeiten1 = berechne_wartezeiten(startzeiten1, endzeiten1, alte_counter(1), counter(1), wartezeiten1);}
  (junction 1094) -> rg1_rot1 : {timer_spuren = countOnwards(timer_spuren,3,[1 0 0 0 1 1 1]);}
  (junction 3449) -> (junction 3435) : {gesamtwartezeit = berechne_gesamtwartezeit(wartezeit_spur1_ges, wartezeit_spur2_ges, wartezeit_spur3_ges, wartezeit_spur4_ges, wartezeit_spur5_ges, wartezeit_spur6_ges, wartezeit_spur7_ges);}
  (junction 3265) -> l1_gelb3 : {timer_spuren = countOnwards(timer_spuren,3,[0 0 1 1 1 1 1]);}
  (junction 3264) -> (junction 3267) : after(5,sec)
      | {timeCounter = refresher(timeCounter, 5);}
  (junction 3453) -> rg1_gelb9 : {timer_spuren = countOnwards(timer_spuren,2,[1 0 0 0 1 1 1]);}
  (junction 1708) -> (junction 1731) : {wartezeit_spur1_ges = gesamt_wartezeit_pro_spur(wartezeiten1, wartezeit_spur1_ges, alte_counter(1), counter(1));}
  Fuss7_rot2 -> (junction 1726) : after(2,sec)
      | {timeCounter = refresher(timeCounter, 2);}
  (junction 3435) -> l1_rot8 : {gesamte_autos = berechne_gesamte_autos(counter(1), counter(2), counter(3), counter(4), counter(5), counter(6), counter(7));}
  l1_gelb3 -> (junction 3260) : after(3,sec)
      | {timeCounter = refresher(timeCounter, 3);}
  (junction 3267) -> Fuss7_rot6 : {timer_spuren = countOnwards(timer_spuren,5,[1 0 0 0 1 1 1]);}
  (junction 1731) -> (junction 1727) : {gesamtwartezeit = berechne_gesamtwartezeit(wartezeit_spur1_ges, wartezeit_spur2_ges, wartezeit_spur3_ges, wartezeit_spur4_ges, wartezeit_spur5_ges, wartezeit_spur6_ges, wartezeit_spur7_ges);}
  ampel2_fuss8_gruen -> (junction 1107) : {[autos_auf_spur3, spur3] = autos_auf_spur_generieren(spur3, gesamtZeit + timeCounter, autos_auf_spur3);}
  rg1_rot1 -> (junction 1124) : {[anz_autos2, autos_auf_spur2, counter(2), endzeiten2] = generiere_gruenphase(2, 50, autos_auf_spur2, counter(2),  (gesamtZeit + timeCounter - 50), endzeiten2, startzeiten2, auslastung, autos_spur1_flag);}
  (junction 3260) -> (junction 3250) : {[autos_auf_spur1, spur1] = autos_auf_spur_generieren(spur1, gesamtZeit + timeCounter, autos_auf_spur1);}
  l1_rot8 -> (junction 3447) : after(3,sec)
      | {timeCounter = refresher(timeCounter, 3);}
  (junction 1726) -> rg1_gelb2 : {timer_spuren = countOnwards(timer_spuren,2,[1 0 0 0 1 1 1]);}
  (junction 1727) -> l1_rot3 : {gesamte_autos = berechne_gesamte_autos(counter(1), counter(2), counter(3), counter(4), counter(5), counter(6), counter(7));}
  rg1_gelb9 -> (junction 3429) : after(3,sec)
      | {timeCounter = refresher(timeCounter, 3);}
  (junction 3447) -> ampel2_rotgelb4 : {timer_spuren = countOnwards(timer_spuren,3,[1 0 1 1 1 1 1]);}
  (junction 1107) -> (junction 1128) : {[autos_auf_spur4, spur4] = autos_auf_spur_generieren(spur4, gesamtZeit + timeCounter, autos_auf_spur4);}
  (junction 3250) -> l1_rot6 : {timer_spuren = countOnwards(timer_spuren,3,[0 0 1 1 1 1 1]);}
  (junction 3429) -> (junction 3428) : {[autos_auf_spur2, spur2] = autos_auf_spur_generieren(spur2, gesamtZeit + timeCounter, autos_auf_spur2);}
  l1_rot3 -> (junction 1728) : after(3,sec)
      | {timeCounter = refresher(timeCounter, 3);}
  (junction 1128) -> (junction 1127) : after(45,sec)
      | {timeCounter = refresher(timeCounter,45);}
  ampel2_rotgelb4 -> (junction 3450) : after(1,sec)
      | {timeCounter = refresher(timeCounter, 1);}
  rg1_gelb2 -> (junction 1732) : after(3,sec)
      | {timeCounter = refresher(timeCounter, 3);}
  l1_rot6 -> (junction 3263) : {[anz_autos1, autos_auf_spur1, counter(1), endzeiten1] = generiere_gruenphase(1, 6, autos_auf_spur1, counter(1),  (gesamtZeit + timeCounter - 6), endzeiten1, startzeiten1, auslastung, autos_spur1_flag);}
  (junction 1728) -> ampel2_rotgelb1 : {timer_spuren = countOnwards(timer_spuren,3,[1 0 1 1 1 1 1]);}
  (junction 1127) -> Fuss7_rot : {timer_spuren = countOnwards(timer_spuren,45,[1 0 0 0 1 1 1]);}
  (junction 3450) -> ampel2_fuss8_gruen4 : {timer_spuren = countOnwards(timer_spuren,1,[1 0 1 1 1 1 1]);}
  (junction 3428) -> rg1_rot23 : {timer_spuren = countOnwards(timer_spuren,3,[1 0 0 0 1 1 1]);}
  (junction 3263) -> (junction 3252) : {wartezeiten1 = berechne_wartezeiten(startzeiten1, endzeiten1, alte_counter(1), counter(1), wartezeiten1);}
  (junction 1732) -> (junction 1706) : {[autos_auf_spur2, spur2] = autos_auf_spur_generieren(spur2, gesamtZeit + timeCounter, autos_auf_spur2);}
  ampel2_rotgelb1 -> (junction 1729) : after(1,sec)
      | {timeCounter = refresher(timeCounter, 1);}
  (junction 1124) -> (junction 1121) : {wartezeiten2 = berechne_wartezeiten(startzeiten2, endzeiten2, alte_counter(2), counter(2), wartezeiten2);}
  (junction 3252) -> (junction 3268) : {wartezeit_spur1_ges = gesamt_wartezeit_pro_spur(wartezeiten1, wartezeit_spur1_ges, alte_counter(1), counter(1));}
  Fuss7_rot6 -> (junction 3261) : after(2,sec)
      | {timeCounter = refresher(timeCounter, 2);}
  (junction 1729) -> ampel2_fuss8_gruen1 : {timer_spuren = countOnwards(timer_spuren,1,[1 0 1 1 1 1 1]);}
  rg1_rot23 -> (junction 3443) : {[anz_autos2, autos_auf_spur2, counter(2), endzeiten2] = generiere_gruenphase(2, 25, autos_auf_spur2, counter(2),  (gesamtZeit + timeCounter - 25), endzeiten2, startzeiten2, auslastung, autos_spur1_flag);}
  (junction 1706) -> rg1_rot6 : {timer_spuren = countOnwards(timer_spuren,3,[1 0 0 0 1 1 1]);}
  (junction 3268) -> (junction 3262) : {gesamtwartezeit = berechne_gesamtwartezeit(wartezeit_spur1_ges, wartezeit_spur2_ges, wartezeit_spur3_ges, wartezeit_spur4_ges, wartezeit_spur5_ges, wartezeit_spur6_ges, wartezeit_spur7_ges);}
  ampel2_fuss8_gruen4 -> (junction 3456) : {[autos_auf_spur3, spur3] = autos_auf_spur_generieren(spur3, gesamtZeit + timeCounter, autos_auf_spur3);}
  (junction 3262) -> l1_rot7 : {gesamte_autos = berechne_gesamte_autos(counter(1), counter(2), counter(3), counter(4), counter(5), counter(6), counter(7));}
  (junction 3261) -> rg1_gelb7 : {timer_spuren = countOnwards(timer_spuren,2,[1 0 0 0 1 1 1]);}
  (junction 3456) -> (junction 3451) : {[autos_auf_spur4, spur4] = autos_auf_spur_generieren(spur4, gesamtZeit + timeCounter, autos_auf_spur4);}
  ampel2_fuss8_gruen1 -> (junction 1733) : {[autos_auf_spur3, spur3] = autos_auf_spur_generieren(spur3, gesamtZeit + timeCounter, autos_auf_spur3);}
  rg1_rot6 -> (junction 1709) : {[anz_autos2, autos_auf_spur2, counter(2), endzeiten2] = generiere_gruenphase(2, 40, autos_auf_spur2, counter(2),  (gesamtZeit + timeCounter - 40), endzeiten2, startzeiten2, auslastung, autos_spur1_flag);}
  Fuss7_rot -> (junction 1114) : after(2,sec)
      | {timeCounter = refresher(timeCounter, 2);}
  (junction 1121) -> (junction 1105) : {wartezeit_spur2_ges = gesamt_wartezeit_pro_spur(wartezeiten2, wartezeit_spur2_ges, alte_counter(2), counter(2));}
  (junction 3451) -> (junction 3440) : after(10,sec)
      | {timeCounter = refresher(timeCounter, 10);}
  l1_rot7 -> (junction 3256) : after(3,sec)
      | {timeCounter = refresher(timeCounter, 3);}
  (junction 1114) -> rg1_gelb : {timer_spuren = countOnwards(timer_spuren,2,[1 0 0 0 1 1 1]);}
  rg1_gelb7 -> (junction 3269) : after(2,sec)
      | {timeCounter = refresher(timeCounter, 2);}
  (junction 1733) -> (junction 1707) : {[autos_auf_spur4, spur4] = autos_auf_spur_generieren(spur4, gesamtZeit + timeCounter, autos_auf_spur4);}
  (junction 3440) -> Fuss7_rot7 : {timer_spuren = countOnwards(timer_spuren,10,[1 0 0 0 1 1 1]);}
  (junction 3256) -> fuss7_rot : {timer_spuren = countOnwards(timer_spuren,3,[1 0 1 1 1 1 1]);}
  (junction 1105) -> (junction 1101) : {gesamtwartezeit = berechne_gesamtwartezeit(wartezeit_spur1_ges, wartezeit_spur2_ges, wartezeit_spur3_ges, wartezeit_spur4_ges, wartezeit_spur5_ges, wartezeit_spur6_ges, wartezeit_spur7_ges)}
  (junction 1707) -> (junction 1713) : after(35,sec)
      | {timeCounter = refresher(timeCounter, 35);}
  (junction 3443) -> (junction 3432) : {wartezeiten2 = berechne_wartezeiten(startzeiten2, endzeiten2, alte_counter(2), counter(2), wartezeiten2);}
  (junction 3269) -> (junction 3266) : {[autos_auf_spur2, spur2] = autos_auf_spur_generieren(spur2, gesamtZeit + timeCounter, autos_auf_spur2);}
  rg1_gelb -> (junction 1100) : after(3,sec)
      | {timeCounter = refresher(timeCounter, 3);}
  (junction 1713) -> Fuss7_rot3 : {timer_spuren = countOnwards(timer_spuren,35,[1 0 0 0 1 1 1]);}
  (junction 1100) -> (junction 1109) : {[autos_auf_spur2, spur2] = autos_auf_spur_generieren(spur2, gesamtZeit + timeCounter, autos_auf_spur2);}
  (junction 3266) -> rg1_rot20 : {timer_spuren = countOnwards(timer_spuren,2,[1 0 0 0 1 1 1]);}
  (junction 1109) -> rg1_rot : {timer_spuren = countOnwards(timer_spuren,3,[1 0 0 0 1 1 1]);}
  (junction 1101) -> rg1_rot5 : {gesamte_autos = berechne_gesamte_autos(counter(1), counter(2), counter(3), counter(4), counter(5), counter(6), counter(7))}
  (junction 1709) -> (junction 1705) : {wartezeiten2 = berechne_wartezeiten(startzeiten2, endzeiten2, alte_counter(2), counter(2), wartezeiten2);}
  fuss7_rot -> (junction 3253) : after(1,sec)
      | {timeCounter = refresher(timeCounter, 1);}
  Fuss7_rot7 -> (junction 3444) : after(2,sec)
      | {timeCounter = refresher(timeCounter, 2);}
  rg1_rot20 -> (junction 3270) : {[anz_autos2, autos_auf_spur2, counter(2), endzeiten2] = generiere_gruenphase(2, 9, autos_auf_spur2, counter(2),  (gesamtZeit + timeCounter - 9), endzeiten2, startzeiten2, auslastung, autos_spur1_flag);}
  (junction 3432) -> (junction 3445) : {wartezeit_spur2_ges = gesamt_wartezeit_pro_spur(wartezeiten2, wartezeit_spur2_ges, alte_counter(2), counter(2));}
  rg1_rot -> (junction 1125) : {[anz_autos2, autos_auf_spur2, counter(2), endzeiten2] = generiere_gruenphase(2, 65, autos_auf_spur2, counter(2),  (gesamtZeit + timeCounter - 65), endzeiten2, startzeiten2, auslastung, autos_spur1_flag);}
  (junction 3253) -> ampel2_rotgelb3 : {timer_spuren = countOnwards(timer_spuren,1,[1 0 1 1 1 1 1]);}
  (junction 3444) -> rg1_gelb8 : {timer_spuren = countOnwards(timer_spuren,2,[1 0 0 0 1 1 1]);}
  Fuss7_rot3 -> (junction 1730) : after(2,sec)
      | {timeCounter = refresher(timeCounter, 2);}
  (junction 1125) -> (junction 1110) : {wartezeiten2 = berechne_wartezeiten(startzeiten2, endzeiten2, alte_counter(2), counter(2), wartezeiten2);}
  (junction 3445) -> (junction 3446) : {gesamtwartezeit = berechne_gesamtwartezeit(wartezeit_spur1_ges, wartezeit_spur2_ges, wartezeit_spur3_ges, wartezeit_spur4_ges, wartezeit_spur5_ges, wartezeit_spur6_ges, wartezeit_spur7_ges)}
  (junction 1705) -> (junction 1716) : {wartezeit_spur2_ges = gesamt_wartezeit_pro_spur(wartezeiten2, wartezeit_spur2_ges, alte_counter(2), counter(2));}
  rg1_rot5 -> (junction 1122)
  rg1_gelb8 -> (junction 3455) : after(3,sec)
      | {timeCounter = refresher(timeCounter, 3);}
  (junction 1730) -> rg1_gelb3 : {timer_spuren = countOnwards(timer_spuren,2,[1 0 0 0 1 1 1]);}
  ampel2_rotgelb3 -> (junction 3251) : after(1,sec)
      | {timeCounter = refresher(timeCounter, 1);}
  (junction 3455) -> (junction 3430) : {[autos_auf_spur2, spur2] = autos_auf_spur_generieren(spur2, gesamtZeit + timeCounter, autos_auf_spur2);}
  (junction 1110) -> (junction 1119) : {wartezeit_spur2_ges = gesamt_wartezeit_pro_spur(wartezeiten2, wartezeit_spur2_ges, alte_counter(2), counter(2));}
  (junction 3251) -> ampel2_fuss8_gruen3 : {timer_spuren = countOnwards(timer_spuren,1,[1 0 1 1 1 1 1]);}
  (junction 1716) -> (junction 1735) : {gesamtwartezeit = berechne_gesamtwartezeit(wartezeit_spur1_ges, wartezeit_spur2_ges, wartezeit_spur3_ges, wartezeit_spur4_ges, wartezeit_spur5_ges, wartezeit_spur6_ges, wartezeit_spur7_ges)}
  (junction 3446) -> fuss8_rot7 : {gesamte_autos = berechne_gesamte_autos(counter(1), counter(2), counter(3), counter(4), counter(5), counter(6), counter(7))}
  (junction 3430) -> rg1_rot26 : {timer_spuren = countOnwards(timer_spuren,3,[1 0 0 0 1 1 1]);}
  rg1_gelb3 -> (junction 1717) : after(3,sec)
      | {timeCounter = refresher(timeCounter, 3);}
  (junction 3270) -> (junction 3255) : {wartezeiten2 = berechne_wartezeiten(startzeiten2, endzeiten2, alte_counter(2), counter(2), wartezeiten2);}
  (junction 1717) -> (junction 1734) : {[autos_auf_spur2, spur2] = autos_auf_spur_generieren(spur2, gesamtZeit + timeCounter, autos_auf_spur2);}
  (junction 1119) -> (junction 1104) : {gesamtwartezeit = berechne_gesamtwartezeit(wartezeit_spur1_ges, wartezeit_spur2_ges, wartezeit_spur3_ges, wartezeit_spur4_ges, wartezeit_spur5_ges, wartezeit_spur6_ges, wartezeit_spur7_ges)}
  rg1_rot26 -> (junction 3425) : {[anz_autos2, autos_auf_spur2, counter(2), endzeiten2] = generiere_gruenphase(2, 30, autos_auf_spur2, counter(2),  (gesamtZeit + timeCounter - 30), endzeiten2, startzeiten2, auslastung, autos_spur1_flag);}
  (junction 1734) -> rg1_rot7 : {timer_spuren = countOnwards(timer_spuren,3,[1 0 0 0 1 1 1]);}
  (junction 1735) -> rg1_rot11 : {gesamte_autos = berechne_gesamte_autos(counter(1), counter(2), counter(3), counter(4), counter(5), counter(6), counter(7))}
  ampel2_fuss8_gruen3 -> (junction 3254) : {[autos_auf_spur3, spur3] = autos_auf_spur_generieren(spur3, gesamtZeit + timeCounter, autos_auf_spur3);}
  (junction 1104) -> rg1_rot4 : {gesamte_autos = berechne_gesamte_autos(counter(1), counter(2), counter(3), counter(4), counter(5), counter(6), counter(7))}
  (junction 3254) -> rg1_gelb6 : {[autos_auf_spur4, spur4] = autos_auf_spur_generieren(spur4, gesamtZeit + timeCounter, autos_auf_spur4);}
  (junction 3425) -> (junction 3427) : {wartezeiten2 = berechne_wartezeiten(startzeiten2, endzeiten2, alte_counter(2), counter(2), wartezeiten2);}
  rg1_rot7 -> (junction 1710) : {[anz_autos2, autos_auf_spur2, counter(2), endzeiten2] = generiere_gruenphase(2, 55, autos_auf_spur2, counter(2),  (gesamtZeit + timeCounter - 55), endzeiten2, startzeiten2, auslastung, autos_spur1_flag);}
  fuss8_rot7 -> (junction 3434)
  (junction 3255) -> (junction 3257) : {wartezeit_spur2_ges = gesamt_wartezeit_pro_spur(wartezeiten2, wartezeit_spur2_ges, alte_counter(2), counter(2));}
  rg1_rot4 -> (junction 1113)
  (junction 3427) -> (junction 3431) : {wartezeit_spur2_ges = gesamt_wartezeit_pro_spur(wartezeiten2, wartezeit_spur2_ges, alte_counter(2), counter(2));}
  (junction 1710) -> (junction 1714) : {wartezeiten2 = berechne_wartezeiten(startzeiten2, endzeiten2, alte_counter(2), counter(2), wartezeiten2);}
  rg1_gelb6 -> (junction 3271) : after(3,sec)
      | {timeCounter = refresher(timeCounter, 3);}
  rg1_rot11 -> (junction 1762)
  (junction 3257) -> (junction 3273) : {gesamtwartezeit = berechne_gesamtwartezeit(wartezeit_spur1_ges, wartezeit_spur2_ges, wartezeit_spur3_ges, wartezeit_spur4_ges, wartezeit_spur5_ges, wartezeit_spur6_ges, wartezeit_spur7_ges)}
  (junction 3271) -> (junction 3272) : {[autos_auf_spur2, spur2] = autos_auf_spur_generieren(spur2, gesamtZeit + timeCounter, autos_auf_spur2);}
  (junction 1714) -> (junction 1718) : {wartezeit_spur2_ges = gesamt_wartezeit_pro_spur(wartezeiten2, wartezeit_spur2_ges, alte_counter(2), counter(2));}
  (junction 3431) -> (junction 3433) : {gesamtwartezeit = berechne_gesamtwartezeit(wartezeit_spur1_ges, wartezeit_spur2_ges, wartezeit_spur3_ges, wartezeit_spur4_ges, wartezeit_spur5_ges, wartezeit_spur6_ges, wartezeit_spur7_ges)}
  (junction 3272) -> rg1_rot17 : {timer_spuren = countOnwards(timer_spuren,3,[1 0 0 0 1 1 1]);}
  (junction 3273) -> fuss8_rot11 : {gesamte_autos = berechne_gesamte_autos(counter(1), counter(2), counter(3), counter(4), counter(5), counter(6), counter(7))}
  rg1_rot17 -> (junction 3104) : {[anz_autos2, autos_auf_spur2, counter(2), endzeiten2] = generiere_gruenphase(2, 13, autos_auf_spur2, counter(2),  (gesamtZeit + timeCounter - 13 ), endzeiten2, startzeiten2, auslastung, autos_spur1_flag);}
  (junction 3433) -> rg1_rot22 : {gesamte_autos = berechne_gesamte_autos(counter(1), counter(2), counter(3), counter(4), counter(5), counter(6), counter(7))}
  (junction 1113) -> (junction 1111)
  (junction 1122) -> (junction 1113)
  (junction 1718) -> (junction 1757) : {gesamtwartezeit = berechne_gesamtwartezeit(wartezeit_spur1_ges, wartezeit_spur2_ges, wartezeit_spur3_ges, wartezeit_spur4_ges, wartezeit_spur5_ges, wartezeit_spur6_ges, wartezeit_spur7_ges)}
  (junction 1111) -> (junction 1112)
  (junction 3104) -> (junction 3101) : {wartezeiten2 = berechne_wartezeiten(startzeiten2, endzeiten2, alte_counter(2), counter(2), wartezeiten2);}
  (junction 1757) -> rg1_rot9 : {gesamte_autos = berechne_gesamte_autos(counter(1), counter(2), counter(3), counter(4), counter(5), counter(6), counter(7))}
  rg1_rot22 -> (junction 3476)
  (junction 3101) -> (junction 3094) : {wartezeit_spur2_ges = gesamt_wartezeit_pro_spur(wartezeiten2, wartezeit_spur2_ges, alte_counter(2), counter(2));}
  fuss8_rot11 -> (junction 3102) : after(2,sec)
      | {timeCounter = refresher(timeCounter, 1);}
  rg1_rot9 -> (junction 1764)
  (junction 3102) -> (junction 3103) : {timer_spuren = countOnwards(timer_spuren,2,[1 1 0 0 1 1 1]);}
  (junction 3094) -> (junction 3096) : {gesamtwartezeit = berechne_gesamtwartezeit(wartezeit_spur1_ges, wartezeit_spur2_ges, wartezeit_spur3_ges, wartezeit_spur4_ges, wartezeit_spur5_ges, wartezeit_spur6_ges, wartezeit_spur7_ges)}
  (junction 3434) -> fuss8_rot13 [order 1] : [autos_auf_spur3 <= 2]
  (junction 3434) -> (junction 3475) [order 2]
  (junction 3436) -> (junction 3528)
  (junction 3476) -> rg1_rot24 [order 1] : [autos_auf_spur3 <= 2]
  (junction 3476) -> (junction 3471) [order 2]
  fuss8_rot13 -> (junction 3469) : %after(2,sec)
      | %{timeCounter = refresher(timeCounter, 2);}
  (junction 3096) -> rg1_rot21 : {gesamte_autos = berechne_gesamte_autos(counter(1), counter(2), counter(3), counter(4), counter(5), counter(6), counter(7))}
  rg1_rot24 -> (junction 3477) : %after(10,sec)
      | %{timeCounter = refresher(timeCounter, 10);}
  (junction 3475) -> fuss8_rot14 [order 1] : [autos_auf_spur3 > 2]
  (junction 3475) -> (junction 3504) [order 2]
  (junction 3471) -> rg1_rot25 [order 1] : [autos_auf_spur3 > 2]
  (junction 3471) -> (junction 3540) [order 2]
  (junction 1764) -> (junction 1741)
  (junction 1762) -> (junction 1764)
  (junction 1741) -> (junction 1751)
  rg1_rot25 -> (junction 3478) : after(15,sec)
      | {timeCounter = refresher(timeCounter, 15);}
  fuss8_rot14 -> (junction 3463) : after(10,sec)
      | {timeCounter = refresher(timeCounter, 10);}
  (junction 3477) -> fuss8_rot5 : %{timer_spuren = countOnwards(timer_spuren,10,[1 1 0 0 1 1 1]);}
  rg1_rot21 -> (junction 3095)
  (junction 3478) -> fuss8_rot4 : {timer_spuren = countOnwards(timer_spuren,15,[1 1 0 0 1 1 1]);}
  fuss8_rot5 -> (junction 3465) : after(2,sec)
      | {timeCounter = refresher(timeCounter, 2);}
  (junction 3469) -> ampel2_gelb12 : %{timer_spuren = countOnwards(timer_spuren,2,[1 1 0 0 1 1 1]);}
  fuss8_rot4 -> (junction 3472) : after(2,sec)
      | {timeCounter = refresher(timeCounter, 2);}
  (junction 3463) -> ampel2_gelb13 : {timer_spuren = countOnwards(timer_spuren,10,[1 1 0 0 1 1 1]);}
  (junction 3465) -> ampel2_gelb5 : {timer_spuren = countOnwards(timer_spuren,2,[1 1 0 0 1 1 1]);}
  (junction 3472) -> ampel2_gelb4 : {timer_spuren = countOnwards(timer_spuren,2,[1 1 0 0 1 1 1]);}
  ampel2_gelb12 -> (junction 3464) : %after(3,sec)
      | %{timeCounter = refresher(timeCounter, 3);}
  (junction 3095) -> rg1_rot19 [order 1] : [autos_auf_spur3 <= 2]
  ampel2_gelb13 -> (junction 3485) : after(3,sec)
      | {timeCounter = refresher(timeCounter, 3);}
  (junction 3095) -> (junction 3097) [order 2]
  (junction 3103) -> ampel2_gelb8 [order 1] : [autos_auf_spur3 <= 2]
  ampel2_gelb5 -> (junction 3483) : after(3,sec)
      | {timeCounter = refresher(timeCounter, 3);}
  (junction 3103) -> (junction 3098) [order 2]
  ampel2_gelb4 -> (junction 3473) : after(3,sec)
      | {timeCounter = refresher(timeCounter, 3);}
  rg1_rot19 -> (junction 3099) : after(3,sec)
      | {timeCounter = refresher(timeCounter, 3);}
  ampel2_gelb8 -> (junction 3118) : after(3,sec)
      | {timeCounter = refresher(timeCounter, 3);}
  (junction 1112) -> rg1_rot3 [order 1] : [autos_auf_spur3 <= 2]
  (junction 3485) -> (junction 3460) : {timer_spuren = countOnwards(timer_spuren,3,[1 1 0 0 1 1 1]);}
  (junction 3464) -> (junction 3480) : %{timer_spuren = countOnwards(timer_spuren,3,[1 1 0 0 1 1 1]);}
  (junction 1112) -> (junction 1115) [order 2]
  (junction 3097) -> rg1_rot18 [order 1] : [autos_auf_spur3 > 2]
  (junction 3473) -> (junction 3467) : {timer_spuren = countOnwards(timer_spuren,3,[1 1 0 0 1 1 1]);}
  (junction 3483) -> (junction 3486) : {timer_spuren = countOnwards(timer_spuren,3,[1 1 0 0 1 1 1]);}
  (junction 3097) -> (junction 3176) [order 2]
  rg1_rot3 -> (junction 1120) : after(7,sec)
      | {timeCounter = refresher(timeCounter, 7);}
  (junction 3098) -> ampel2_gelb11 [order 1] : [autos_auf_spur3 > 2]
  rg1_rot18 -> (junction 3100) : after(3,sec)
      | {timeCounter = refresher(timeCounter, 3);}
  (junction 3098) -> (junction 3184) [order 2]
  (junction 1115) -> rg1_rot2 [order 1] : [autos_auf_spur3 > 2]
  ampel2_gelb11 -> (junction 3117) : after(3,sec)
      | {timeCounter = refresher(timeCounter, 3);}
  (junction 1115) -> (junction 1138) [order 2]
  (junction 3099) -> fuss8_rot10 : {timer_spuren = countOnwards(timer_spuren,3,[1 1 0 0 1 1 1]);}
  (junction 3460) -> (junction 3470) : {[autos_auf_spur3, spur3] = autos_auf_spur_generieren(spur3, gesamtZeit + timeCounter, autos_auf_spur3);}
  (junction 3480) -> (junction 3474) : {[autos_auf_spur3, spur3] = autos_auf_spur_generieren(spur3, gesamtZeit + timeCounter, autos_auf_spur3);}
  rg1_rot2 -> (junction 1116) : after(20,sec)
      | {timeCounter = refresher(timeCounter, 20);}
  (junction 3467) -> (junction 3466) : {[autos_auf_spur3, spur3] = autos_auf_spur_generieren(spur3, gesamtZeit + timeCounter, autos_auf_spur3);}
  (junction 3486) -> (junction 3459) : {[autos_auf_spur3, spur3] = autos_auf_spur_generieren(spur3, gesamtZeit + timeCounter, autos_auf_spur3);}
  (junction 1120) -> fuss8_rot1 : {timer_spuren = countOnwards(timer_spuren,7,[1 1 0 0 1 1 1]);}
  (junction 3470) -> ampel2_rot24 : {[autos_auf_spur4, spur4] = autos_auf_spur_generieren(spur4, gesamtZeit + timeCounter, autos_auf_spur4);}
  (junction 3100) -> fuss8_rot12 : {timer_spuren = countOnwards(timer_spuren,3,[1 1 0 0 1 1 1]);}
  (junction 3466) -> ampel2_rot11 : {[autos_auf_spur4, spur4] = autos_auf_spur_generieren(spur4, gesamtZeit + timeCounter, autos_auf_spur4);}
  (junction 3474) -> ampel2_rot25 : {[autos_auf_spur4, spur4] = autos_auf_spur_generieren(spur4, gesamtZeit + timeCounter, autos_auf_spur4);}
  (junction 3459) -> ampel2_rot9 : {[autos_auf_spur4, spur4] = autos_auf_spur_generieren(spur4, gesamtZeit + timeCounter, autos_auf_spur4);}
  (junction 1116) -> fuss8_rot : {timer_spuren = countOnwards(timer_spuren,20,[1 1 0 0 1 1 1]);}
  fuss8_rot10 -> (junction 3127) : after(2,sec)
      | {timeCounter = refresher(timeCounter, 2);}
  ampel2_rot24 -> (junction 3481) : {[anz_autos3, autos_auf_spur3, counter(3), endzeiten3] = generiere_gruenphase(3, 40, autos_auf_spur3, counter(3),  (gesamtZeit + timeCounter - 40), endzeiten3, startzeiten3, auslastung, autos_spur1_flag)}
  ampel2_rot11 -> (junction 3479) : {[anz_autos3, autos_auf_spur3, counter(3), endzeiten3] = generiere_gruenphase(3, 35, autos_auf_spur3, counter(3),  (gesamtZeit + timeCounter -  35), endzeiten3, startzeiten3, auslastung, autos_spur1_flag)}
  fuss8_rot12 -> (junction 3107) : after(2,sec)
      | {timeCounter = refresher(timeCounter, 2);}
  fuss8_rot1 -> (junction 1106) : after(2,sec)
      | {timeCounter = refresher(timeCounter, 2);}
  (junction 3127) -> ampel2_gelb9 : {timer_spuren = countOnwards(timer_spuren,2,[1 1 0 0 1 1 1]);}
  (junction 3107) -> ampel2_gelb10 : {timer_spuren = countOnwards(timer_spuren,2,[1 1 0 0 1 1 1]);}
  fuss8_rot -> (junction 1108) : after(2,sec)
      | {timeCounter = refresher(timeCounter, 2);}
  (junction 1106) -> ampel2_gelb1 : {timer_spuren = countOnwards(timer_spuren,2,[1 1 0 0 1 1 1]);}
  (junction 1108) -> ampel2_gelb : {timer_spuren = countOnwards(timer_spuren,2,[1 1 0 0 1 1 1]);}
  (junction 3481) -> (junction 3462) : {wartezeiten3 = berechne_wartezeiten(startzeiten3, endzeiten3, alte_counter(3), counter(3), wartezeiten3);}
  ampel2_gelb9 -> (junction 3112) : after(3,sec)
      | {timeCounter = refresher(timeCounter, 3);}
  ampel2_gelb10 -> (junction 3124) : after(3,sec)
      | {timeCounter = refresher(timeCounter, 3);}
  (junction 1751) -> rg1_rot8 [order 1] : [autos_auf_spur3 <= 2]
  (junction 3479) -> (junction 3482) : {wartezeiten3 = berechne_wartezeiten(startzeiten3, endzeiten3, alte_counter(3), counter(3), wartezeiten3);}
  (junction 1751) -> (junction 1742) [order 2]
  ampel2_gelb1 -> (junction 1130) : after(3,sec)
      | {timeCounter = refresher(timeCounter, 3);}
  (junction 3124) -> (junction 3125) : {timer_spuren = countOnwards(timer_spuren,3,[1 1 0 0 1 1 1]);}
  (junction 3112) -> (junction 3113) : {timer_spuren = countOnwards(timer_spuren,3,[1 1 0 0 1 1 1]);}
  rg1_rot8 -> (junction 1744) : after(7,sec)
      | {timeCounter = refresher(timeCounter, 7);}
  ampel2_gelb -> (junction 1129) : after(3,sec)
      | {timeCounter = refresher(timeCounter, 3);}
  (junction 1742) -> rg1_rot10 [order 1] : [autos_auf_spur3 > 2]
  (junction 3117) -> (junction 3126) : {timer_spuren = countOnwards(timer_spuren,3,[1 1 0 0 1 1 1]);}
  (junction 3118) -> (junction 3114) : {timer_spuren = countOnwards(timer_spuren,3,[1 1 0 0 1 1 1]);}
  (junction 3462) -> (junction 3484) : {wartezeit_spur3_ges = gesamt_wartezeit_pro_spur(wartezeiten3, wartezeit_spur3_ges, alte_counter(3), counter(3));}
  (junction 1742) -> (junction 1768) [order 2]
  (junction 1129) -> (junction 1126) : {timer_spuren = countOnwards(timer_spuren,3,[1 1 0 0 1 1 1]);}
  (junction 1130) -> (junction 1123) : {timer_spuren = countOnwards(timer_spuren,3,[1 1 0 0 1 1 1]);}
  (junction 3482) -> (junction 3457) : {wartezeit_spur3_ges = gesamt_wartezeit_pro_spur(wartezeiten3, wartezeit_spur3_ges, alte_counter(3), counter(3));}
  rg1_rot10 -> (junction 1739) : after(20,sec)
      | {timeCounter = refresher(timeCounter, 20);}
  ampel2_rot25 -> (junction 3487) : {[anz_autos3, autos_auf_spur3, counter(3), endzeiten3] = generiere_gruenphase(3, 25, autos_auf_spur3, counter(3),  (gesamtZeit + timeCounter - 25), endzeiten3, startzeiten3, auslastung, autos_spur1_flag)}
  (junction 3125) -> (junction 3119) : {[autos_auf_spur3, spur3] = autos_auf_spur_generieren(spur3, gesamtZeit + timeCounter, autos_auf_spur3);}
  (junction 3113) -> (junction 3115) : {[autos_auf_spur3, spur3] = autos_auf_spur_generieren(spur3, gesamtZeit + timeCounter, autos_auf_spur3);}
  (junction 1744) -> fuss8_rot3 : {timer_spuren = countOnwards(timer_spuren,7,[1 1 0 0 1 1 1]);}
  ampel2_rot9 -> (junction 3458) : {[anz_autos3, autos_auf_spur3, counter(3), endzeiten3] = generiere_gruenphase(3, 20, autos_auf_spur3, counter(3),  (gesamtZeit + timeCounter - 20), endzeiten3, startzeiten3, auslastung, autos_spur1_flag)}
  (junction 3126) -> (junction 3106) : {[autos_auf_spur3, spur3] = autos_auf_spur_generieren(spur3, gesamtZeit + timeCounter, autos_auf_spur3);}
  (junction 3114) -> (junction 3111) : {[autos_auf_spur3, spur3] = autos_auf_spur_generieren(spur3, gesamtZeit + timeCounter, autos_auf_spur3);}
  (junction 1126) -> (junction 1117) : {[autos_auf_spur3, spur3] = autos_auf_spur_generieren(spur3, gesamtZeit + timeCounter, autos_auf_spur3);}
  (junction 1123) -> (junction 1118) : {[autos_auf_spur3, spur3] = autos_auf_spur_generieren(spur3, gesamtZeit + timeCounter, autos_auf_spur3);}
  (junction 3484) -> (junction 3461) : {gesamtwartezeit = berechne_gesamtwartezeit(wartezeit_spur1_ges, wartezeit_spur2_ges, wartezeit_spur3_ges, wartezeit_spur4_ges, wartezeit_spur5_ges, wartezeit_spur6_ges, wartezeit_spur7_ges);}
  (junction 3119) -> ampel2_rot19 : {[autos_auf_spur4, spur4] = autos_auf_spur_generieren(spur4, gesamtZeit + timeCounter, autos_auf_spur4);}
  (junction 3120) -> (junction 3108)
  (junction 3487) -> (junction 3517) : {wartezeiten3 = berechne_wartezeiten(startzeiten3, endzeiten3, alte_counter(3), counter(3), wartezeiten3);}
  (junction 3457) -> (junction 3468) : {gesamtwartezeit = berechne_gesamtwartezeit(wartezeit_spur1_ges, wartezeit_spur2_ges, wartezeit_spur3_ges, wartezeit_spur4_ges, wartezeit_spur5_ges, wartezeit_spur6_ges, wartezeit_spur7_ges);}
  (junction 1739) -> fuss8_rot2 : {timer_spuren = countOnwards(timer_spuren,20,[1 1 0 0 1 1 1]);}
  (junction 3458) -> (junction 3506) : {wartezeiten3 = berechne_wartezeiten(startzeiten3, endzeiten3, alte_counter(3), counter(3), wartezeiten3);}
  (junction 3106) -> ampel2_rot17 : {[autos_auf_spur4, spur4] = autos_auf_spur_generieren(spur4, gesamtZeit + timeCounter, autos_auf_spur4);}
  (junction 3115) -> ampel2_rot21 : {[autos_auf_spur4, spur4] = autos_auf_spur_generieren(spur4, gesamtZeit + timeCounter, autos_auf_spur4);}
  (junction 1117) -> ampel2_rot : {[autos_auf_spur4, spur4] = autos_auf_spur_generieren(spur4, gesamtZeit + timeCounter, autos_auf_spur4);}
  (junction 3111) -> ampel2_rot20 : {[autos_auf_spur4, spur4] = autos_auf_spur_generieren(spur4, gesamtZeit + timeCounter, autos_auf_spur4);}
  (junction 3461) -> (junction 3516) : {gesamte_autos = berechne_gesamte_autos(counter(1), counter(2), counter(3), counter(4), counter(5), counter(6), counter(7));}
  (junction 1118) -> ampel2_rot1 : {[autos_auf_spur4, spur4] = autos_auf_spur_generieren(spur4, gesamtZeit + timeCounter, autos_auf_spur4);}
  (junction 3468) -> (junction 3518) : {gesamte_autos = berechne_gesamte_autos(counter(1), counter(2), counter(3), counter(4), counter(5), counter(6), counter(7));}
  (junction 3517) -> (junction 3505) : {wartezeit_spur3_ges = gesamt_wartezeit_pro_spur(wartezeiten3, wartezeit_spur3_ges, alte_counter(3), counter(3));}
  ampel2_rot19 -> (junction 3109) : {[anz_autos3, autos_auf_spur3, counter(3), endzeiten3] = generiere_gruenphase(3, 11, autos_auf_spur3, counter(3),  (gesamtZeit + timeCounter - 11), endzeiten3, startzeiten3, auslastung, autos_spur1_flag);}
  fuss8_rot3 -> (junction 1738) : after(2,sec)
      | {timeCounter = refresher(timeCounter, 2);}
  (junction 3506) -> (junction 3491) : {wartezeit_spur3_ges = gesamt_wartezeit_pro_spur(wartezeiten3, wartezeit_spur3_ges, alte_counter(3), counter(3));}
  ampel2_rot17 -> (junction 3123) : {[anz_autos3, autos_auf_spur3, counter(3), endzeiten3] = generiere_gruenphase(3, 14, autos_auf_spur3, counter(3),  (gesamtZeit + timeCounter - 14), endzeiten3, startzeiten3, auslastung, autos_spur1_flag);}
  fuss8_rot2 -> (junction 1748) : after(2,sec)
      | {timeCounter = refresher(timeCounter, 2);}
  (junction 3108) -> (junction 3121)
  ampel2_rot -> (junction 1102) : {[anz_autos3, autos_auf_spur3, counter(3), endzeiten3] = generiere_gruenphase(3, 75, autos_auf_spur3, counter(3),  (gesamtZeit + timeCounter - 75), endzeiten3, startzeiten3, auslastung, autos_spur1_flag);}
  (junction 3516) -> (junction 3492) : {[anz_autos4, autos_auf_spur4, counter(4), endzeiten4] = generiere_gruenphase(4, 40, autos_auf_spur4, counter(4),  (gesamtZeit + timeCounter - 40), endzeiten4, startzeiten4, autos_spur1_flag)}
  (junction 1738) -> ampel2_gelb3 : {timer_spuren = countOnwards(timer_spuren,2,[1 1 0 0 1 1 1]);}
  (junction 3518) -> (junction 3489) : {[anz_autos4, autos_auf_spur4, counter(4), endzeiten4] = generiere_gruenphase(4, 35, autos_auf_spur4, counter(4),  (gesamtZeit + timeCounter - 35), endzeiten4, startzeiten4, autos_spur1_flag)}
  (junction 1748) -> ampel2_gelb2 : {timer_spuren = countOnwards(timer_spuren,2,[1 1 0 0 1 1 1]);}
  (junction 3505) -> (junction 3509) : {gesamtwartezeit = berechne_gesamtwartezeit(wartezeit_spur1_ges, wartezeit_spur2_ges, wartezeit_spur3_ges, wartezeit_spur4_ges, wartezeit_spur5_ges, wartezeit_spur6_ges, wartezeit_spur7_ges);}
  (junction 3121) -> (junction 3186)
  (junction 3491) -> (junction 3500) : {gesamtwartezeit = berechne_gesamtwartezeit(wartezeit_spur1_ges, wartezeit_spur2_ges, wartezeit_spur3_ges, wartezeit_spur4_ges, wartezeit_spur5_ges, wartezeit_spur6_ges, wartezeit_spur7_ges)}
  (junction 3492) -> (junction 3519) : {wartezeiten4 = berechne_wartezeiten(startzeiten4, endzeiten4, alte_counter(4), counter(4), wartezeiten4);}
  (junction 3109) -> (junction 3122) : {wartezeiten3 = berechne_wartezeiten(startzeiten3, endzeiten3, alte_counter(3), counter(3), wartezeiten3);}
  ampel2_gelb3 -> (junction 1765) : after(3,sec)
      | {timeCounter = refresher(timeCounter, 3);}
  (junction 3489) -> (junction 3515) : {wartezeiten4 = berechne_wartezeiten(startzeiten4, endzeiten4, alte_counter(4), counter(4), wartezeiten4);}
  ampel2_gelb2 -> (junction 1746) : after(3,sec)
      | {timeCounter = refresher(timeCounter, 3);}
  (junction 3123) -> (junction 3110) : {wartezeiten3 = berechne_wartezeiten(startzeiten3, endzeiten3, alte_counter(3), counter(3), wartezeiten3);}
  (junction 1102) -> (junction 1131) : {wartezeiten3 = berechne_wartezeiten(startzeiten3, endzeiten3, alte_counter(3), counter(3), wartezeiten3);}
  (junction 3509) -> (junction 3498) : {gesamte_autos = berechne_gesamte_autos(counter(1), counter(2), counter(3), counter(4), counter(5), counter(6), counter(7));}
  (junction 1746) -> (junction 1760) : {timer_spuren = countOnwards(timer_spuren,3,[1 1 0 0 1 1 1]);}
  (junction 1765) -> (junction 1758) : {timer_spuren = countOnwards(timer_spuren,3,[1 1 0 0 1 1 1]);}
  (junction 3500) -> (junction 3513) : {gesamte_autos = berechne_gesamte_autos(counter(1), counter(2), counter(3), counter(4), counter(5), counter(6), counter(7));}
  (junction 3519) -> (junction 3507) : {wartezeit_spur4_ges = gesamt_wartezeit_pro_spur(wartezeiten4, wartezeit_spur4_ges, alte_counter(4), counter(4));}
  (junction 3498) -> (junction 3520) : {[anz_autos4, autos_auf_spur4, counter(4), endzeiten4] = generiere_gruenphase(4, 25, autos_auf_spur4, counter(4),  (gesamtZeit + timeCounter - 25), endzeiten4, startzeiten4, auslastung, autos_spur1_flag)}
  (junction 3122) -> (junction 3116) : {wartezeit_spur3_ges = gesamt_wartezeit_pro_spur(wartezeiten3, wartezeit_spur3_ges, alte_counter(3), counter(3));}
  (junction 3515) -> (junction 3501) : {wartezeit_spur4_ges = gesamt_wartezeit_pro_spur(wartezeiten4, wartezeit_spur4_ges, alte_counter(4), counter(4));}
  (junction 3513) -> (junction 3493) : {[anz_autos4, autos_auf_spur4, counter(4), endzeiten4] = generiere_gruenphase(4, 20, autos_auf_spur4, counter(4),  (gesamtZeit + timeCounter - 20), endzeiten4, startzeiten4, auslastung, autos_spur1_flag);}
  (junction 3110) -> (junction 3147) : {wartezeit_spur3_ges = gesamt_wartezeit_pro_spur(wartezeiten3, wartezeit_spur3_ges, alte_counter(3), counter(3));}
  ampel2_rot21 -> (junction 3105) : {[anz_autos3, autos_auf_spur3, counter(3), endzeiten3] = generiere_gruenphase(3, 11, autos_auf_spur3, counter(3),  (gesamtZeit + timeCounter - 11), endzeiten3, startzeiten3, auslastung, autos_spur1_flag);}
  (junction 1131) -> (junction 1103) : {wartezeit_spur3_ges = gesamt_wartezeit_pro_spur(wartezeiten3, wartezeit_spur3_ges, alte_counter(3), counter(3));}
  (junction 3520) -> (junction 3508) : {wartezeiten4 = berechne_wartezeiten(startzeiten4, endzeiten4, alte_counter(4), counter(4), wartezeiten4);}
  (junction 1760) -> (junction 1753) : {[autos_auf_spur3, spur3] = autos_auf_spur_generieren(spur3, gesamtZeit + timeCounter, autos_auf_spur3);}
  (junction 1758) -> (junction 1743) : {[autos_auf_spur3, spur3] = autos_auf_spur_generieren(spur3, gesamtZeit + timeCounter, autos_auf_spur3);}
  ampel2_rot20 -> (junction 3153) : {[anz_autos3, autos_auf_spur3, counter(3), endzeiten3] = generiere_gruenphase(3, 14, autos_auf_spur3, counter(3),  (gesamtZeit + timeCounter - 14), endzeiten3, startzeiten3, auslastung, autos_spur1_flag);}
  (junction 3493) -> (junction 3499) : {wartezeiten4 = berechne_wartezeiten(startzeiten4, endzeiten4, alte_counter(4), counter(4), wartezeiten4);}
  ampel2_rot1 -> (junction 1158) : {[anz_autos3, autos_auf_spur3, counter(3), endzeiten3] = generiere_gruenphase(3, 62, autos_auf_spur3, counter(3),  (gesamtZeit + timeCounter - 62), endzeiten3, startzeiten3, auslastung, autos_spur1_flag);}
  (junction 3507) -> (junction 3502) : {gesamtwartezeit = berechne_gesamtwartezeit(wartezeit_spur1_ges, wartezeit_spur2_ges, wartezeit_spur3_ges, wartezeit_spur4_ges, wartezeit_spur5_ges, wartezeit_spur6_ges, wartezeit_spur7_ges);}
  (junction 3116) -> (junction 3136) : {gesamtwartezeit = berechne_gesamtwartezeit(wartezeit_spur1_ges, wartezeit_spur2_ges, wartezeit_spur3_ges, wartezeit_spur4_ges, wartezeit_spur5_ges, wartezeit_spur6_ges, wartezeit_spur7_ges);}
  (junction 3105) -> (junction 3139) : {wartezeiten3 = berechne_wartezeiten(startzeiten3, endzeiten3, alte_counter(3), counter(3), wartezeiten3);}
  (junction 1753) -> ampel2_rot5 : {[autos_auf_spur4, spur4] = autos_auf_spur_generieren(spur4, gesamtZeit + timeCounter, autos_auf_spur4);}
  (junction 3501) -> (junction 3488) : {gesamtwartezeit = berechne_gesamtwartezeit(wartezeit_spur1_ges, wartezeit_spur2_ges, wartezeit_spur3_ges, wartezeit_spur4_ges, wartezeit_spur5_ges, wartezeit_spur6_ges, wartezeit_spur7_ges);}
  (junction 3508) -> (junction 3514) : {wartezeit_spur4_ges = gesamt_wartezeit_pro_spur(wartezeiten4, wartezeit_spur4_ges, alte_counter(4), counter(4));}
  (junction 3147) -> (junction 3140) : {gesamtwartezeit = berechne_gesamtwartezeit(wartezeit_spur1_ges, wartezeit_spur2_ges, wartezeit_spur3_ges, wartezeit_spur4_ges, wartezeit_spur5_ges, wartezeit_spur6_ges, wartezeit_spur7_ges);}
  (junction 1103) -> (junction 1143) : {gesamtwartezeit = berechne_gesamtwartezeit(wartezeit_spur1_ges, wartezeit_spur2_ges, wartezeit_spur3_ges, wartezeit_spur4_ges, wartezeit_spur5_ges, wartezeit_spur6_ges, wartezeit_spur7_ges);}
  (junction 3153) -> (junction 3156) : {wartezeiten3 = berechne_wartezeiten(startzeiten3, endzeiten3, alte_counter(3), counter(3), wartezeiten3);}
  (junction 1743) -> ampel2_rot6 : {[autos_auf_spur4, spur4] = autos_auf_spur_generieren(spur4, gesamtZeit + timeCounter, autos_auf_spur4);}
  (junction 3499) -> (junction 3490) : {wartezeit_spur4_ges = gesamt_wartezeit_pro_spur(wartezeiten4, wartezeit_spur4_ges, alte_counter(4), counter(4));}
  (junction 1158) -> (junction 1153) : {wartezeiten3 = berechne_wartezeiten(startzeiten3, endzeiten3, alte_counter(3), counter(3), wartezeiten3);}
  (junction 3502) -> ampel2_rot26 : {gesamte_autos = berechne_gesamte_autos(counter(1), counter(2), counter(3), counter(4), counter(5), counter(6), counter(7));}
  (junction 3136) -> (junction 3152) : {gesamte_autos = berechne_gesamte_autos(counter(1), counter(2), counter(3), counter(4), counter(5), counter(6), counter(7));}
  (junction 3514) -> (junction 3511) : {gesamtwartezeit = berechne_gesamtwartezeit(wartezeit_spur1_ges, wartezeit_spur2_ges, wartezeit_spur3_ges, wartezeit_spur4_ges, wartezeit_spur5_ges, wartezeit_spur6_ges, wartezeit_spur7_ges);}
  (junction 3488) -> ampel2_rot10 : {gesamte_autos = berechne_gesamte_autos(counter(1), counter(2), counter(3), counter(4), counter(5), counter(6), counter(7));}
  (junction 3139) -> (junction 3142) : {wartezeit_spur3_ges = gesamt_wartezeit_pro_spur(wartezeiten3, wartezeit_spur3_ges, alte_counter(3), counter(3));}
  (junction 3140) -> (junction 3128) : {gesamte_autos = berechne_gesamte_autos(counter(1), counter(2), counter(3), counter(4), counter(5), counter(6), counter(7));}
  ampel2_rot5 -> (junction 1747) : {[anz_autos3, autos_auf_spur3, counter(3), endzeiten3] = generiere_gruenphase(3, 65, autos_auf_spur3, counter(3),  (gesamtZeit + timeCounter - 65), endzeiten3, startzeiten3, auslastung, autos_spur1_flag);}
  (junction 3490) -> (junction 3494) : {gesamtwartezeit = berechne_gesamtwartezeit(wartezeit_spur1_ges, wartezeit_spur2_ges, wartezeit_spur3_ges, wartezeit_spur4_ges, wartezeit_spur5_ges, wartezeit_spur6_ges, wartezeit_spur7_ges);}
  (junction 1143) -> (junction 1137) : {gesamte_autos = berechne_gesamte_autos(counter(1), counter(2), counter(3), counter(4), counter(5), counter(6), counter(7));}
  (junction 3156) -> (junction 3129) : {wartezeit_spur3_ges = gesamt_wartezeit_pro_spur(wartezeiten3, wartezeit_spur3_ges, alte_counter(3), counter(3));}
  (junction 1153) -> (junction 1144) : {wartezeit_spur3_ges = gesamt_wartezeit_pro_spur(wartezeiten3, wartezeit_spur3_ges, alte_counter(3), counter(3));}
  (junction 3152) -> (junction 3131) : {[anz_autos4, autos_auf_spur4, counter(4), endzeiten4] = generiere_gruenphase(4, 55, autos_auf_spur4, counter(4),  (gesamtZeit + timeCounter -55), endzeiten4, startzeiten4, autos_spur1_flag);}
  (junction 3511) -> ampel2_rot27 : {gesamte_autos = berechne_gesamte_autos(counter(1), counter(2), counter(3), counter(4), counter(5), counter(6), counter(7));}
  (junction 3494) -> ampel2_rot8 : {gesamte_autos = berechne_gesamte_autos(counter(1), counter(2), counter(3), counter(4), counter(5), counter(6), counter(7));}
  (junction 3128) -> (junction 3143) : {[anz_autos4, autos_auf_spur4, counter(4), endzeiten4] = generiere_gruenphase(4, 55, autos_auf_spur4, counter(4),  (gesamtZeit + timeCounter -55), endzeiten4, startzeiten4, autos_spur1_flag);}
  (junction 1137) -> (junction 1147) : {[anz_autos4, autos_auf_spur4, counter(4), endzeiten4] = generiere_gruenphase(4, 75, autos_auf_spur4, counter(4),  (gesamtZeit + timeCounter - 75), endzeiten4, startzeiten4, autos_spur1_flag);}
  (junction 3142) -> (junction 3145) : {gesamtwartezeit = berechne_gesamtwartezeit(wartezeit_spur1_ges, wartezeit_spur2_ges, wartezeit_spur3_ges, wartezeit_spur4_ges, wartezeit_spur5_ges, wartezeit_spur6_ges, wartezeit_spur7_ges);}
  ampel2_rot26 -> (junction 3496) : after(1,sec)
      | {timeCounter = refresher(timeCounter, 1);}
  (junction 3131) -> (junction 3154) : {wartezeiten4 = berechne_wartezeiten(startzeiten4, endzeiten4, alte_counter(4), counter(4), wartezeiten4);}
  (junction 3129) -> (junction 3155) : {gesamtwartezeit = berechne_gesamtwartezeit(wartezeit_spur1_ges, wartezeit_spur2_ges, wartezeit_spur3_ges, wartezeit_spur4_ges, wartezeit_spur5_ges, wartezeit_spur6_ges, wartezeit_spur7_ges);}
  (junction 1747) -> (junction 1759) : {wartezeiten3 = berechne_wartezeiten(startzeiten3, endzeiten3, alte_counter(3), counter(3), wartezeiten3);}
  (junction 1144) -> (junction 1156) : {gesamtwartezeit = berechne_gesamtwartezeit(wartezeit_spur1_ges, wartezeit_spur2_ges, wartezeit_spur3_ges, wartezeit_spur4_ges, wartezeit_spur5_ges, wartezeit_spur6_ges, wartezeit_spur7_ges);}
  ampel2_rot10 -> (junction 3495) : after(1,sec)
      | {timeCounter = refresher(timeCounter, 1);}
  (junction 3143) -> (junction 3132) : {wartezeiten4 = berechne_wartezeiten(startzeiten4, endzeiten4, alte_counter(4), counter(4), wartezeiten4);}
  ampel2_rot27 -> (junction 3510) : after(1,sec)
      | {timeCounter = refresher(timeCounter, 1);}
  (junction 1147) -> (junction 1146) : {wartezeiten4 = berechne_wartezeiten(startzeiten4, endzeiten4, alte_counter(4), counter(4), wartezeiten4);}
  (junction 3145) -> (junction 3157) : {gesamte_autos = berechne_gesamte_autos(counter(1), counter(2), counter(3), counter(4), counter(5), counter(6), counter(7));}
  (junction 3496) -> rg3_rotgelb13 : {timer_spuren = countOnwards(timer_spuren,1,[1 1 1 1 1 1 1]);}
  ampel2_rot8 -> (junction 3503) : after(1,sec)
      | {timeCounter = refresher(timeCounter, 1);}
  (junction 3495) -> rg3_rotgelb4 : {timer_spuren = countOnwards(timer_spuren,1,[1 1 1 1 1 1 1]);}
  (junction 3155) -> (junction 3146) : {gesamte_autos = berechne_gesamte_autos(counter(1), counter(2), counter(3), counter(4), counter(5), counter(6), counter(7));}
  (junction 3510) -> rg3_rotgelb14 : {timer_spuren = countOnwards(timer_spuren,1,[1 1 1 1 1 1 1]);}
  (junction 3154) -> (junction 3144) : {wartezeit_spur4_ges = gesamt_wartezeit_pro_spur(wartezeiten4, wartezeit_spur4_ges, alte_counter(4), counter(4));}
  (junction 3157) -> (junction 3149) : {[anz_autos4, autos_auf_spur4, counter(4), endzeiten4] = generiere_gruenphase(4, 42, autos_auf_spur4, counter(4),  (gesamtZeit + timeCounter -42), endzeiten4, startzeiten4, auslastung, autos_spur1_flag);}
  (junction 1156) -> (junction 1148) : {gesamte_autos = berechne_gesamte_autos(counter(1), counter(2), counter(3), counter(4), counter(5), counter(6), counter(7));}
  (junction 1759) -> (junction 1756) : {wartezeit_spur3_ges = gesamt_wartezeit_pro_spur(wartezeiten3, wartezeit_spur3_ges, alte_counter(3), counter(3));}
  (junction 3503) -> rg3_rotgelb5 : {timer_spuren = countOnwards(timer_spuren,1,[1 1 1 1 1 1 1]);}
  rg3_rotgelb13 -> (junction 3512)
  (junction 3132) -> (junction 3159) : {wartezeit_spur4_ges = gesamt_wartezeit_pro_spur(wartezeiten4, wartezeit_spur4_ges, alte_counter(4), counter(4));}
  (junction 3146) -> (junction 3148) : {[anz_autos4, autos_auf_spur4, counter(4), endzeiten4] = generiere_gruenphase(4, 42, autos_auf_spur4, counter(4),  (gesamtZeit + timeCounter -42), endzeiten4, startzeiten4, auslastung, autos_spur1_flag);}
  (junction 1146) -> (junction 1149) : {wartezeit_spur4_ges = gesamt_wartezeit_pro_spur(wartezeiten4, wartezeit_spur4_ges, alte_counter(4), counter(4));}
  (junction 1148) -> (junction 1155) : {[anz_autos4, autos_auf_spur4, counter(4), endzeiten4] = generiere_gruenphase(4, 62, autos_auf_spur4, counter(4),  (gesamtZeit + timeCounter - 62), endzeiten4, startzeiten4, auslastung, autos_spur1_flag);}
  rg3_rotgelb4 -> (junction 3548)
  ampel2_rot6 -> (junction 1737) : {[anz_autos3, autos_auf_spur3, counter(3), endzeiten3] = generiere_gruenphase(3, 52, autos_auf_spur3, counter(3),  (gesamtZeit + timeCounter - 52), endzeiten3, startzeiten3, auslastung, autos_spur1_flag);}
  (junction 3149) -> (junction 3133) : {wartezeiten4 = berechne_wartezeiten(startzeiten4, endzeiten4, alte_counter(4), counter(4), wartezeiten4);}
  rg3_rotgelb14 -> (junction 3497)
  (junction 3148) -> (junction 3158) : {wartezeiten4 = berechne_wartezeiten(startzeiten4, endzeiten4, alte_counter(4), counter(4), wartezeiten4);}
  (junction 3512) -> (junction 3504)
  (junction 3497) -> (junction 3512)
  rg3_rotgelb5 -> (junction 3552)
  (junction 3144) -> (junction 3138) : {gesamtwartezeit = berechne_gesamtwartezeit(wartezeit_spur1_ges, wartezeit_spur2_ges, wartezeit_spur3_ges, wartezeit_spur4_ges, wartezeit_spur5_ges, wartezeit_spur6_ges, wartezeit_spur7_ges);}
  (junction 3504) -> (junction 3532)
  (junction 1155) -> (junction 1140) : {wartezeiten4 = berechne_wartezeiten(startzeiten4, endzeiten4, alte_counter(4), counter(4), wartezeiten4);}
  (junction 1756) -> (junction 1740) : {gesamtwartezeit = berechne_gesamtwartezeit(wartezeit_spur1_ges, wartezeit_spur2_ges, wartezeit_spur3_ges, wartezeit_spur4_ges, wartezeit_spur5_ges, wartezeit_spur6_ges, wartezeit_spur7_ges);}
  (junction 3548) -> (junction 3540)
  (junction 3552) -> (junction 3548)
  (junction 3540) -> (junction 3535)
  (junction 1737) -> (junction 1761) : {wartezeiten3 = berechne_wartezeiten(startzeiten3, endzeiten3, alte_counter(3), counter(3), wartezeiten3);}
  (junction 3159) -> (junction 3141) : {gesamtwartezeit = berechne_gesamtwartezeit(wartezeit_spur1_ges, wartezeit_spur2_ges, wartezeit_spur3_ges, wartezeit_spur4_ges, wartezeit_spur5_ges, wartezeit_spur6_ges, wartezeit_spur7_ges);}
  (junction 3133) -> (junction 3130) : {wartezeit_spur4_ges = gesamt_wartezeit_pro_spur(wartezeiten4, wartezeit_spur4_ges, alte_counter(4), counter(4));}
  (junction 1149) -> (junction 1157) : {gesamtwartezeit = berechne_gesamtwartezeit(wartezeit_spur1_ges, wartezeit_spur2_ges, wartezeit_spur3_ges, wartezeit_spur4_ges, wartezeit_spur5_ges, wartezeit_spur6_ges, wartezeit_spur7_ges);}
  (junction 3158) -> (junction 3134) : {wartezeit_spur4_ges = gesamt_wartezeit_pro_spur(wartezeiten4, wartezeit_spur4_ges, alte_counter(4), counter(4));}
  (junction 1140) -> (junction 1136) : {wartezeit_spur4_ges = gesamt_wartezeit_pro_spur(wartezeiten4, wartezeit_spur4_ges, alte_counter(4), counter(4));}
  (junction 3138) -> ampel2_rot16 : {gesamte_autos = berechne_gesamte_autos(counter(1), counter(2), counter(3), counter(4), counter(5), counter(6), counter(7));}
  (junction 1740) -> (junction 1749) : {gesamte_autos = berechne_gesamte_autos(counter(1), counter(2), counter(3), counter(4), counter(5), counter(6), counter(7));}
  (junction 3130) -> (junction 3135) : {gesamtwartezeit = berechne_gesamtwartezeit(wartezeit_spur1_ges, wartezeit_spur2_ges, wartezeit_spur3_ges, wartezeit_spur4_ges, wartezeit_spur5_ges, wartezeit_spur6_ges, wartezeit_spur7_ges);}
  (junction 3141) -> ampel2_rot22 : {gesamte_autos = berechne_gesamte_autos(counter(1), counter(2), counter(3), counter(4), counter(5), counter(6), counter(7));}
  (junction 1761) -> (junction 1750) : {wartezeit_spur3_ges = gesamt_wartezeit_pro_spur(wartezeiten3, wartezeit_spur3_ges, alte_counter(3), counter(3));}
  (junction 1157) -> ampel2_rot2 : {gesamte_autos = berechne_gesamte_autos(counter(1), counter(2), counter(3), counter(4), counter(5), counter(6), counter(7));}
  (junction 3134) -> (junction 3150) : {gesamtwartezeit = berechne_gesamtwartezeit(wartezeit_spur1_ges, wartezeit_spur2_ges, wartezeit_spur3_ges, wartezeit_spur4_ges, wartezeit_spur5_ges, wartezeit_spur6_ges, wartezeit_spur7_ges);}
  (junction 1136) -> (junction 1141) : {gesamtwartezeit = berechne_gesamtwartezeit(wartezeit_spur1_ges, wartezeit_spur2_ges, wartezeit_spur3_ges, wartezeit_spur4_ges, wartezeit_spur5_ges, wartezeit_spur6_ges, wartezeit_spur7_ges);}
  (junction 3135) -> ampel2_rot18 : {gesamte_autos = berechne_gesamte_autos(counter(1), counter(2), counter(3), counter(4), counter(5), counter(6), counter(7));}
  (junction 1749) -> (junction 1752) : {[anz_autos4, autos_auf_spur4, counter(4), endzeiten4] = generiere_gruenphase(4, 65, autos_auf_spur4, counter(4),  (gesamtZeit + timeCounter - 65), endzeiten4, startzeiten4, autos_spur1_flag);}
  (junction 3150) -> ampel2_rot23 : {gesamte_autos = berechne_gesamte_autos(counter(1), counter(2), counter(3), counter(4), counter(5), counter(6), counter(7));}
  (junction 1141) -> ampel2_rot3 : {gesamte_autos = berechne_gesamte_autos(counter(1), counter(2), counter(3), counter(4), counter(5), counter(6), counter(7));}
  (junction 1750) -> (junction 1763) : {gesamtwartezeit = berechne_gesamtwartezeit(wartezeit_spur1_ges, wartezeit_spur2_ges, wartezeit_spur3_ges, wartezeit_spur4_ges, wartezeit_spur5_ges, wartezeit_spur6_ges, wartezeit_spur7_ges);}
  ampel2_rot16 -> (junction 3137) : after(1,sec)
      | {timeCounter = refresher(timeCounter, 1);}
  (junction 1752) -> (junction 1766) : {wartezeiten4 = berechne_wartezeiten(startzeiten4, endzeiten4, alte_counter(4), counter(4), wartezeiten4);}
  (junction 3535) -> (junction 3528)
  (junction 3532) -> (junction 3535)
  ampel2_rot22 -> (junction 3170) : after(1,sec)
      | {timeCounter = refresher(timeCounter, 1);}
  (junction 3528) -> (junction 3537) : {[autos_auf_spur5, spur5] = autos_auf_spur_generieren(spur5, gesamtZeit + timeCounter, autos_auf_spur5);}
  ampel2_rot18 -> (junction 3151) : after(1,sec)
      | {timeCounter = refresher(timeCounter, 1);}
  ampel2_rot2 -> (junction 1142) : after(1,sec)
      | {timeCounter = refresher(timeCounter, 1);}
  (junction 3137) -> rg3_rotgelb10 : {timer_spuren = countOnwards(timer_spuren,1,[1 1 1 1 1 1 1]);}
  (junction 1763) -> (junction 1745) : {gesamte_autos = berechne_gesamte_autos(counter(1), counter(2), counter(3), counter(4), counter(5), counter(6), counter(7));}
  ampel2_rot23 -> (junction 3174) : after(1,sec)
      | {timeCounter = refresher(timeCounter, 1);}
  ampel2_rot3 -> (junction 1163) : after(1,sec)
      | {timeCounter = refresher(timeCounter, 1);}
  (junction 3151) -> rg3_rotgelb12 : {timer_spuren = countOnwards(timer_spuren,1,[1 1 1 1 1 1 1]);}
  (junction 3170) -> rg3_rotgelb11 : {timer_spuren = countOnwards(timer_spuren,1,[1 1 1 1 1 1 1]);}
  (junction 1766) -> (junction 1754) : {wartezeit_spur4_ges = gesamt_wartezeit_pro_spur(wartezeiten4, wartezeit_spur4_ges, alte_counter(4), counter(4));}
  (junction 1745) -> (junction 1736) : {[anz_autos4, autos_auf_spur4, counter(4), endzeiten4] = generiere_gruenphase(4, 52, autos_auf_spur4, counter(4),  (gesamtZeit + timeCounter - 52), endzeiten4, startzeiten4, auslastung, autos_spur1_flag);}
  (junction 1142) -> rg3_rotgelb : {timer_spuren = countOnwards(timer_spuren,1,[1 1 1 1 1 1 1]);}
  (junction 3174) -> rg3_rotgelb9 : {timer_spuren = countOnwards(timer_spuren,1,[1 1 1 1 1 1 1]);}
  rg3_rotgelb10 -> (junction 3183)
  (junction 1163) -> rg3_rotgelb1 : {timer_spuren = countOnwards(timer_spuren,1,[1 1 1 1 1 1 1]);}
  rg3_rotgelb11 -> (junction 3172)
  (junction 1736) -> (junction 1755) : {wartezeiten4 = berechne_wartezeiten(startzeiten4, endzeiten4, alte_counter(4), counter(4), wartezeiten4);}
  rg3_rotgelb12 -> (junction 3171)
  rg3_rotgelb -> (junction 1133)
  (junction 3183) -> (junction 3176)
  (junction 3171) -> (junction 3183)
  (junction 3176) -> (junction 3161)
  rg3_rotgelb9 -> (junction 3175)
  (junction 1754) -> (junction 1777) : {gesamtwartezeit = berechne_gesamtwartezeit(wartezeit_spur1_ges, wartezeit_spur2_ges, wartezeit_spur3_ges, wartezeit_spur4_ges, wartezeit_spur5_ges, wartezeit_spur6_ges, wartezeit_spur7_ges);}
  rg3_rotgelb1 -> (junction 1150)
  (junction 3172) -> (junction 3184)
  (junction 3175) -> (junction 3172)
  (junction 3184) -> (junction 3166)
  (junction 1133) -> (junction 1138)
  (junction 1150) -> (junction 1133)
  (junction 1755) -> (junction 1769) : {wartezeit_spur4_ges = gesamt_wartezeit_pro_spur(wartezeiten4, wartezeit_spur4_ges, alte_counter(4), counter(4));}
  (junction 1138) -> (junction 1151) : {[autos_auf_spur5, spur5] = autos_auf_spur_generieren(spur5, gesamtZeit + timeCounter, autos_auf_spur5);}
  (junction 1777) -> ampel2_rot7 : {gesamte_autos = berechne_gesamte_autos(counter(1), counter(2), counter(3), counter(4), counter(5), counter(6), counter(7));}
  (junction 1769) -> (junction 1791) : {gesamtwartezeit = berechne_gesamtwartezeit(wartezeit_spur1_ges, wartezeit_spur2_ges, wartezeit_spur3_ges, wartezeit_spur4_ges, wartezeit_spur5_ges, wartezeit_spur6_ges, wartezeit_spur7_ges);}
  (junction 1791) -> ampel2_rot4 : {gesamte_autos = berechne_gesamte_autos(counter(1), counter(2), counter(3), counter(4), counter(5), counter(6), counter(7));}
  (junction 1151) -> (junction 1154) [order 1] : [autos_auf_spur5 == 0]
  (junction 1151) -> (junction 1139) [order 2]
  (junction 1154) -> (junction 1160) : after(1,sec)
      | {timeCounter = refresher(timeCounter, 1);}
  (junction 3161) -> (junction 3186)
  (junction 3166) -> (junction 3161)
  (junction 3186) -> (junction 3177) : {[autos_auf_spur5, spur5] = autos_auf_spur_generieren(spur5, gesamtZeit + timeCounter, autos_auf_spur5);}
  ampel2_rot7 -> (junction 1775) : after(1,sec)
      | {timeCounter = refresher(timeCounter, 1);}
  (junction 1139) -> (junction 1159) [order 1] : [autos_auf_spur5 > 0]
  (junction 1139) -> (junction 1184) [order 2]
  (junction 1159) -> l3_rotgelb_rg3_fuss6_gruen
  ampel2_rot4 -> (junction 1799) : after(1,sec)
      | {timeCounter = refresher(timeCounter, 1);}
  (junction 1775) -> rg3_rotgelb2 : {timer_spuren = countOnwards(timer_spuren,1,[1 1 1 1 1 1 1]);}
  (junction 1160) -> rg3_fuss6_gruen : {timer_spuren = countOnwards(timer_spuren,1,[1 1 1 1 1 1 1]);}
  (junction 1799) -> rg3_rotgelb3 : {timer_spuren = countOnwards(timer_spuren,1,[1 1 1 1 1 1 1]);}
  rg3_rotgelb2 -> (junction 1776)
  rg3_rotgelb3 -> (junction 1792)
  (junction 1776) -> (junction 1768)
  (junction 1792) -> (junction 1776)
  l3_rotgelb_rg3_fuss6_gruen -> (junction 1162) : {[autos_auf_spur6, spur6] = autos_auf_spur_generieren(spur6, gesamtZeit + timeCounter, autos_auf_spur6);}
  rg3_fuss6_gruen -> (junction 1132) : {[autos_auf_spur6, spur6] = autos_auf_spur_generieren(spur6, gesamtZeit + timeCounter, autos_auf_spur6);}
  (junction 1768) -> (junction 1783) : {[autos_auf_spur5, spur5] = autos_auf_spur_generieren(spur5, gesamtZeit + timeCounter, autos_auf_spur5);}
  (junction 1132) -> (junction 1161) : after(4,sec)
      | {timeCounter = refresher(timeCounter, 4);}
  (junction 1162) -> (junction 1152) : after(1,sec)
      | {timeCounter = refresher(timeCounter, 1);}
  (junction 3537) -> rg3_rotgelb6 [order 1] : [autos_auf_spur5 == 0]
  (junction 3537) -> (junction 3525) [order 2]
  rg3_rotgelb6 -> (junction 3547) : after(1,sec)
      | {timeCounter = refresher(timeCounter, 1);}
  (junction 1152) -> l3_gruen : {timer_spuren = countOnwards(timer_spuren,1,[1 1 1 1 1 0 1]);}
  (junction 1161) -> ampel4_rotgelb : {timer_spuren = countOnwards(timer_spuren,4,[1 1 1 1 1 0 1]);}
  (junction 3525) -> (junction 3530) [order 1] : [autos_auf_spur5 > 0]
  (junction 3525) -> (junction 3563) [order 2]
  (junction 3530) -> l3_rotgelb_rg3_fuss6_gruen4
  (junction 1783) -> (junction 1770) [order 1] : [autos_auf_spur5 == 0]
  (junction 3547) -> rg3_fuss6_gruen4 : {timer_spuren = countOnwards(timer_spuren,1,[1 1 1 1 1 1 1]);}
  (junction 1783) -> (junction 1797) [order 2]
  (junction 1770) -> (junction 1767) : after(1,sec)
      | {timeCounter = refresher(timeCounter, 1);}
  ampel4_rotgelb -> (junction 1134) : after(1,sec)
      | {timeCounter = refresher(timeCounter, 1);}
  (junction 1797) -> (junction 1793) [order 1] : [autos_auf_spur5 > 0]
  (junction 1797) -> (junction 1800) [order 2]
  (junction 1793) -> l3_rotgelb_rg3_fuss6_gruen1
  l3_gruen -> (junction 1135) : after(8,sec)
      | {timeCounter = refresher(timeCounter, 8);}
  (junction 1767) -> rg3_fuss6_gruen1 : {timer_spuren = countOnwards(timer_spuren,1,[1 1 1 1 1 1 1]);}
  l3_rotgelb_rg3_fuss6_gruen4 -> (junction 3531) : {[autos_auf_spur6, spur6] = autos_auf_spur_generieren(spur6, gesamtZeit + timeCounter, autos_auf_spur6);}
  rg3_fuss6_gruen4 -> (junction 3523) : {[autos_auf_spur6, spur6] = autos_auf_spur_generieren(spur6, gesamtZeit + timeCounter, autos_auf_spur6);}
  (junction 1134) -> ampel4_fuss5_gruen : {timer_spuren = countOnwards(timer_spuren,1,[1 1 1 1 1 0 1]);}
  (junction 3523) -> (junction 3521) : after(4,sec)
      | {timeCounter = refresher(timeCounter, 4);}
  (junction 3531) -> (junction 3536) : after(1,sec)
      | {timeCounter = refresher(timeCounter, 1);}
  (junction 1135) -> l3_gelb : {timer_spuren = countOnwards(timer_spuren,8,[1 1 1 1 0 0 1]);}
  l3_rotgelb_rg3_fuss6_gruen1 -> (junction 1794) : {[autos_auf_spur6, spur6] = autos_auf_spur_generieren(spur6, gesamtZeit + timeCounter, autos_auf_spur6);}
  rg3_fuss6_gruen1 -> (junction 1771) : {[autos_auf_spur6, spur6] = autos_auf_spur_generieren(spur6, gesamtZeit + timeCounter, autos_auf_spur6);}
  (junction 3536) -> l3_gruen4 : {timer_spuren = countOnwards(timer_spuren,1,[1 1 1 1 1 0 1]);}
  (junction 3521) -> ampel4_rotgelb4 : {timer_spuren = countOnwards(timer_spuren,4,[1 1 1 1 1 0 1]);}
  (junction 1771) -> (junction 1784) : after(4,sec)
      | {timeCounter = refresher(timeCounter, 4);}
  (junction 1794) -> (junction 1786) : after(1,sec)
      | {timeCounter = refresher(timeCounter, 1);}
  (junction 3177) -> (junction 3182) [order 1] : [autos_auf_spur5 == 0]
  (junction 3177) -> (junction 3173) [order 2]
  (junction 3182) -> (junction 3178) : after(1,sec)
      | {timeCounter = refresher(timeCounter, 1);}
  ampel4_rotgelb4 -> (junction 3522) : after(1,sec)
      | {timeCounter = refresher(timeCounter, 1);}
  (junction 1786) -> l3_gruen1 : {timer_spuren = countOnwards(timer_spuren,1,[1 1 1 1 1 0 1]);}
  (junction 1784) -> ampel4_rotgelb1 : {timer_spuren = countOnwards(timer_spuren,4,[1 1 1 1 1 0 1]);}
  (junction 3173) -> (junction 3187) [order 1] : [autos_auf_spur5 > 0]
  (junction 3173) -> (junction 3203) [order 2]
  (junction 3187) -> l3_rotgelb_rg3_fuss6_gruen3
  l3_gelb -> (junction 1145) : after(3,sec)
      | {timeCounter = refresher(timeCounter, 3);}
  l3_gruen4 -> (junction 3549) : after(6,sec)
      | {timeCounter = refresher(timeCounter, 6);}
  (junction 3178) -> rg3_fuss6_gruen3 : {timer_spuren = countOnwards(timer_spuren,1,[1 1 1 1 1 1 1]);}
  (junction 1145) -> (junction 1172) : {timer_spuren = countOnwards(timer_spuren,3,[1 1 1 1 0 0 1]);}
  ampel4_rotgelb1 -> (junction 1787) : after(1,sec)
      | {timeCounter = refresher(timeCounter, 1);}
  (junction 3522) -> ampel4_fuss5_gruen8 : {timer_spuren = countOnwards(timer_spuren,1,[1 1 1 1 1 0 1]);}
  l3_gruen1 -> (junction 1795) : after(8,sec)
      | {timeCounter = refresher(timeCounter, 8);}
  (junction 1172) -> l3_fuss6_rot : {[autos_auf_spur5, spur5] = autos_auf_spur_generieren(spur5, gesamtZeit + timeCounter, autos_auf_spur5);}
  (junction 3549) -> l3_gelb_fuss6_rot : {timer_spuren = countOnwards(timer_spuren,6,[1 1 1 1 0 0 1]);}
  ampel4_fuss5_gruen -> (junction 1190) : {[autos_auf_spur7, spur7] = autos_auf_spur_generieren(spur7, gesamtZeit + timeCounter, autos_auf_spur7);}
  l3_rotgelb_rg3_fuss6_gruen3 -> (junction 3160) : {[autos_auf_spur6, spur6] = autos_auf_spur_generieren(spur6, gesamtZeit + timeCounter, autos_auf_spur6);}
  rg3_fuss6_gruen3 -> (junction 3167) : {[autos_auf_spur6, spur6] = autos_auf_spur_generieren(spur6, gesamtZeit + timeCounter, autos_auf_spur6);}
  (junction 1787) -> ampel4_fuss5_gruen2 : {timer_spuren = countOnwards(timer_spuren,1,[1 1 1 1 1 0 1]);}
  (junction 1190) -> (junction 1176) : after(6,sec)
      | {timeCounter = refresher(timeCounter, 6);}
  (junction 3167) -> (junction 3168) : after(4,sec)
      | {timeCounter = refresher(timeCounter, 4);}
  (junction 1795) -> l3_gelb1 : {timer_spuren = countOnwards(timer_spuren,8,[1 1 1 1 0 0 1]);}
  (junction 3160) -> (junction 3162) : after(1,sec)
      | {timeCounter = refresher(timeCounter, 1);}
  l3_fuss6_rot -> (junction 1171) : {[anz_autos5, autos_auf_spur5, counter(5), endzeiten5] = generiere_gruenphase(5, 11, autos_auf_spur5, counter(5),  (gesamtZeit + timeCounter -11), endzeiten5, startzeiten5, auslastung, autos_spur1_flag);}
  l3_gelb_fuss6_rot -> (junction 3545) : after(1,sec)
      | {timeCounter = refresher(timeCounter, 1);}
  (junction 3162) -> l3_gruen3 : {timer_spuren = countOnwards(timer_spuren,1,[1 1 1 1 1 0 1]);}
  (junction 3168) -> ampel4_rotgelb3 : {timer_spuren = countOnwards(timer_spuren,4,[1 1 1 1 1 0 1]);}
  (junction 3545) -> (junction 3538) : {timer_spuren = countOnwards(timer_spuren,1,[1 1 1 1 0 0 1]);}
  ampel4_rotgelb3 -> (junction 3185) : after(1,sec)
      | {timeCounter = refresher(timeCounter, 1);}
  (junction 1171) -> (junction 1193) : {wartezeiten5 = berechne_wartezeiten(startzeiten5, endzeiten5, alte_counter(5), counter(5), wartezeiten5);}
  (junction 3538) -> fuss6_rot6 : {[autos_auf_spur5, spur5] = autos_auf_spur_generieren(spur5, gesamtZeit + timeCounter, autos_auf_spur5);}
  l3_gelb1 -> (junction 1798) : after(3,sec)
      | {timeCounter = refresher(timeCounter, 3);}
  l3_gruen3 -> (junction 3180) : after(3,sec)
      | {timeCounter = refresher(timeCounter, 3);}
  ampel4_fuss5_gruen8 -> (junction 3527) : {[autos_auf_spur7, spur7] = autos_auf_spur_generieren(spur7, gesamtZeit + timeCounter, autos_auf_spur7);}
  (junction 1798) -> (junction 1785) : {timer_spuren = countOnwards(timer_spuren,3,[1 1 1 1 0 0 1]);}
  fuss6_rot6 -> (junction 3539) : after(2,sec)
      | {timeCounter = refresher(timeCounter, 2);}
  (junction 1193) -> (junction 1166) : {wartezeit_spur5_ges = gesamt_wartezeit_pro_spur(wartezeiten5, wartezeit_spur5_ges, alte_counter(5), counter(5));}
  (junction 3185) -> ampel4_fuss5_gruen6 : {timer_spuren = countOnwards(timer_spuren,1,[1 1 1 1 1 0 1]);}
  (junction 1785) -> l3_fuss6_rot3 : {[autos_auf_spur5, spur5] = autos_auf_spur_generieren(spur5, gesamtZeit + timeCounter, autos_auf_spur5);}
  (junction 3527) -> (junction 3541) : after(2,sec)
      | {timeCounter = refresher(timeCounter, 2);}
  (junction 3180) -> l3_gelb2 : {timer_spuren = countOnwards(timer_spuren,3,[1 1 1 1 0 0 1]);}
  ampel4_fuss5_gruen2 -> (junction 1772) : {[autos_auf_spur7, spur7] = autos_auf_spur_generieren(spur7, gesamtZeit + timeCounter, autos_auf_spur7);}
  (junction 3539) -> l3_rot1 : {timer_spuren = countOnwards(timer_spuren,2,[1 1 1 1 0 0 1]);}
  (junction 1166) -> (junction 1164) : {gesamtwartezeit = berechne_gesamtwartezeit(wartezeit_spur1_ges, wartezeit_spur2_ges, wartezeit_spur3_ges, wartezeit_spur4_ges, wartezeit_spur5_ges, wartezeit_spur6_ges, wartezeit_spur7_ges);}
  (junction 1772) -> (junction 1780) : after(6,sec)
      | {timeCounter = refresher(timeCounter, 6);}
  (junction 1164) -> l3_fuss6_rot1 : {gesamte_autos = berechne_gesamte_autos(counter(1), counter(2), counter(3), counter(4), counter(5), counter(6), counter(7));}
  l3_fuss6_rot3 -> (junction 1796) : {[anz_autos5, autos_auf_spur5, counter(5), endzeiten5] = generiere_gruenphase(5, 11, autos_auf_spur5, counter(5),  (gesamtZeit + timeCounter -11), endzeiten5, startzeiten5, auslastung, autos_spur1_flag);}
  l3_rot1 -> (junction 3526) : {[anz_autos5, autos_auf_spur5, counter(5), endzeiten5] = generiere_gruenphase(5, 9, autos_auf_spur5, counter(5),  (gesamtZeit + timeCounter - 9), endzeiten5, startzeiten5, auslastung, autos_spur1_flag);}
  (junction 1176) -> fuss6_rot : {timer_spuren = countOnwards(timer_spuren,6,[1 1 1 1 1 0 0]);}
  (junction 3526) -> (junction 3533) : {wartezeiten5 = berechne_wartezeiten(startzeiten5, endzeiten5, alte_counter(5), counter(5), wartezeiten5);}
  l3_gelb2 -> fuss6_rot4 : after(1,sec)
      | {timeCounter = refresher(timeCounter, 1);}
  l3_fuss6_rot1 -> (junction 1179) : after(2,sec)
      | {timeCounter = refresher(timeCounter, 2);}
  (junction 3533) -> (junction 3524) : {wartezeit_spur5_ges = gesamt_wartezeit_pro_spur(wartezeiten5, wartezeit_spur5_ges, alte_counter(5), counter(5));}
  (junction 1796) -> (junction 1773) : {wartezeiten5 = berechne_wartezeiten(startzeiten5, endzeiten5, alte_counter(5), counter(5), wartezeiten5);}
  fuss6_rot -> (junction 1186) : after(2,sec)
      | {timeCounter = refresher(timeCounter, 2);}
  fuss6_rot4 -> (junction 3163) : after(2,sec)
      | {timeCounter = refresher(timeCounter, 2);}
  (junction 1179) -> rg3_gelb1 : {timer_spuren = countOnwards(timer_spuren,2,[1 1 1 1 1 0 1]);}
  ampel4_fuss5_gruen6 -> fuss6_rot5 : {[autos_auf_spur7, spur7] = autos_auf_spur_generieren(spur7, gesamtZeit + timeCounter, autos_auf_spur7);}
  (junction 1186) -> rg3_gelb : {timer_spuren = countOnwards(timer_spuren,2,[1 1 1 1 1 0 0]);}
  (junction 1773) -> (junction 1774) : {wartezeit_spur5_ges = gesamt_wartezeit_pro_spur(wartezeiten5, wartezeit_spur5_ges, alte_counter(5), counter(5));}
  (junction 3524) -> (junction 3529) : {gesamtwartezeit = berechne_gesamtwartezeit(wartezeit_spur1_ges, wartezeit_spur2_ges, wartezeit_spur3_ges, wartezeit_spur4_ges, wartezeit_spur5_ges, wartezeit_spur6_ges, wartezeit_spur7_ges);}
  (junction 3163) -> (junction 3164) : {timer_spuren = countOnwards(timer_spuren,3,[1 1 1 1 0 0 1]);}
  (junction 3164) -> l3_rot_rg3_gelb : {[autos_auf_spur5, spur5] = autos_auf_spur_generieren(spur5, gesamtZeit + timeCounter, autos_auf_spur5);}
  (junction 3529) -> l3_rot : {gesamte_autos = berechne_gesamte_autos(counter(1), counter(2), counter(3), counter(4), counter(5), counter(6), counter(7));}
  rg3_gelb1 -> (junction 1169) : after(3,sec)
      | {timeCounter = refresher(timeCounter, 3);}
  rg3_gelb -> (junction 1188) : after(3,sec)
      | {timeCounter = refresher(timeCounter, 3);}
  (junction 1774) -> (junction 1779) : {gesamtwartezeit = berechne_gesamtwartezeit(wartezeit_spur1_ges, wartezeit_spur2_ges, wartezeit_spur3_ges, wartezeit_spur4_ges, wartezeit_spur5_ges, wartezeit_spur6_ges, wartezeit_spur7_ges);}
  (junction 3541) -> fuss6_rot7 : {timer_spuren = countOnwards(timer_spuren,2,[1 1 1 1 1 0 0]);}
  (junction 1779) -> l3_fuss6_rot2 : {gesamte_autos = berechne_gesamte_autos(counter(1), counter(2), counter(3), counter(4), counter(5), counter(6), counter(7));}
  (junction 1169) -> (junction 1189) : {timer_spuren = countOnwards(timer_spuren,3,[1 1 1 1 1 0 1]);}
  l3_rot_rg3_gelb -> (junction 3165) : {[anz_autos5, autos_auf_spur5, counter(5), endzeiten5] = generiere_gruenphase(5, 6, autos_auf_spur5, counter(5),  (gesamtZeit + timeCounter - 6), endzeiten5, startzeiten5, auslastung, autos_spur1_flag);}
  l3_rot -> (junction 3534) : %after(2,sec)
      | %{timeCounter = refresher(timeCounter, 2);}
  (junction 1188) -> (junction 1194) : {timer_spuren = countOnwards(timer_spuren,3,[1 1 1 1 1 0 0]);}
  (junction 1780) -> fuss6_rot1 : {timer_spuren = countOnwards(timer_spuren,6,[1 1 1 1 1 0 0]);}
  (junction 3165) -> (junction 3190) : {wartezeiten5 = berechne_wartezeiten(startzeiten5, endzeiten5, alte_counter(5), counter(5), wartezeiten5);}
  (junction 1189) -> rg3_rot_ampel4_rotgelb : {[autos_auf_spur6, spur6] = autos_auf_spur_generieren(spur6, gesamtZeit + timeCounter, autos_auf_spur6);}
  fuss6_rot7 -> (junction 3546) : after(2,sec)
      | {timeCounter = refresher(timeCounter, 2);}
  (junction 3534) -> rg3_gelb8 : %{timer_spuren = countOnwards(timer_spuren,2,[1 1 1 1 1 0 1]);}
  (junction 3546) -> rg3_gelb7 : {timer_spuren = countOnwards(timer_spuren,2,[1 1 1 1 1 0 0]);}
  l3_fuss6_rot2 -> (junction 1778) : after(2,sec)
      | {timeCounter = refresher(timeCounter, 2);}
  (junction 3190) -> (junction 3179) : {wartezeit_spur5_ges = gesamt_wartezeit_pro_spur(wartezeiten5, wartezeit_spur5_ges, alte_counter(5), counter(5));}
  fuss6_rot1 -> (junction 1781) : after(2,sec)
      | {timeCounter = refresher(timeCounter, 2);}
  (junction 1778) -> rg3_gelb2 : {timer_spuren = countOnwards(timer_spuren,2,[1 1 1 1 1 0 1]);}
  rg3_gelb8 -> (junction 3543) : after(3,sec)
      | {timeCounter = refresher(timeCounter, 3);}
  rg3_gelb7 -> (junction 3542) : after(3,sec)
      | {timeCounter = refresher(timeCounter, 3);}
  (junction 1781) -> rg3_gelb3 : {timer_spuren = countOnwards(timer_spuren,2,[1 1 1 1 1 0 0]);}
  (junction 1194) -> rg3_fuss5_rot : {[autos_auf_spur6, spur6] = autos_auf_spur_generieren(spur6, gesamtZeit + timeCounter, autos_auf_spur6);}
  (junction 3179) -> (junction 3188) : {gesamtwartezeit = berechne_gesamtwartezeit(wartezeit_spur1_ges, wartezeit_spur2_ges, wartezeit_spur3_ges, wartezeit_spur4_ges, wartezeit_spur5_ges, wartezeit_spur6_ges, wartezeit_spur7_ges);}
  rg3_rot_ampel4_rotgelb -> (junction 1192) : {[anz_autos6, autos_auf_spur6, counter(6), endzeiten6] = generiere_gruenphase(6, 17, autos_auf_spur6, counter(6),  (gesamtZeit + timeCounter -17), endzeiten6, startzeiten6, auslastung, autos_spur1_flag);}
  (junction 3543) -> (junction 3544) : {timer_spuren = countOnwards(timer_spuren,3,[1 1 1 1 1 0 1]);}
  (junction 3188) -> l3_rot_rg3_gelb1 : {gesamte_autos = berechne_gesamte_autos(counter(1), counter(2), counter(3), counter(4), counter(5), counter(6), counter(7));}
  rg3_gelb2 -> (junction 1782) : after(3,sec)
      | {timeCounter = refresher(timeCounter, 3);}
  rg3_gelb3 -> (junction 1788) : after(3,sec)
      | {timeCounter = refresher(timeCounter, 3);}
  (junction 3542) -> (junction 3550) : {timer_spuren = countOnwards(timer_spuren,3,[1 1 1 1 1 0 0]);}
  (junction 3544) -> rg3_rot_ampel4_rotgelb8 : {[autos_auf_spur6, spur6] = autos_auf_spur_generieren(spur6, gesamtZeit + timeCounter, autos_auf_spur6);}
  (junction 1782) -> (junction 1789) : {timer_spuren = countOnwards(timer_spuren,3,[1 1 1 1 1 0 1]);}
  (junction 1192) -> (junction 1182) : {wartezeiten6 = berechne_wartezeiten(startzeiten6, endzeiten6, alte_counter(6), counter(6), wartezeiten6);}
  (junction 1788) -> (junction 1790) : {timer_spuren = countOnwards(timer_spuren,3,[1 1 1 1 1 0 0]);}
  rg3_fuss5_rot -> (junction 1185) : {[anz_autos6, autos_auf_spur6, counter(6), endzeiten6] = generiere_gruenphase(6, 17, autos_auf_spur6, counter(6),  (gesamtZeit + timeCounter -17), endzeiten6, startzeiten6, auslastung, autos_spur1_flag);}
  (junction 1789) -> rg3_rot_ampel4_rotgelb2 : {[autos_auf_spur6, spur6] = autos_auf_spur_generieren(spur6, gesamtZeit + timeCounter, autos_auf_spur6);}
  fuss6_rot5 -> (junction 3181) : after(2,sec)
      | {timeCounter = refresher(timeCounter, 2);}
  (junction 1182) -> (junction 1177) : {wartezeit_spur6_ges = gesamt_wartezeit_pro_spur(wartezeiten6, wartezeit_spur6_ges, alte_counter(6), counter(6));}
  (junction 3550) -> rg3_fuss5_rot8 : {[autos_auf_spur6, spur6] = autos_auf_spur_generieren(spur6, gesamtZeit + timeCounter, autos_auf_spur6);}
  (junction 3181) -> rg3_gelb6 : {timer_spuren = countOnwards(timer_spuren,2,[1 1 1 1 1 0 0]);}
  rg3_rot_ampel4_rotgelb8 -> (junction 3551) : {[anz_autos6, autos_auf_spur6, counter(6), endzeiten6] = generiere_gruenphase(6, 12, autos_auf_spur6, counter(6),  (gesamtZeit + timeCounter - 12), endzeiten6, startzeiten6, auslastung, autos_spur1_flag);}
  l3_rot_rg3_gelb1 -> (junction 3189) : after(3,sec)
      | {timeCounter = refresher(timeCounter, 3);}
  (junction 1177) -> (junction 1191) : {gesamtwartezeit = berechne_gesamtwartezeit(wartezeit_spur1_ges, wartezeit_spur2_ges, wartezeit_spur3_ges, wartezeit_spur4_ges, wartezeit_spur5_ges, wartezeit_spur6_ges, wartezeit_spur7_ges);}
  (junction 1790) -> rg3_fuss5_rot2 : {[autos_auf_spur6, spur6] = autos_auf_spur_generieren(spur6, gesamtZeit + timeCounter, autos_auf_spur6);}
  rg3_gelb6 -> (junction 3169) : after(1,sec)
      | {timeCounter = refresher(timeCounter, 1);}
  rg3_rot_ampel4_rotgelb2 -> (junction 1826) : {[anz_autos6, autos_auf_spur6, counter(6), endzeiten6] = generiere_gruenphase(6, 17, autos_auf_spur6, counter(6),  (gesamtZeit + timeCounter -17), endzeiten6, startzeiten6, auslastung, autos_spur1_flag);}
  (junction 1191) -> rg3_rot_ampel4_rotgelb1 : {gesamte_autos = berechne_gesamte_autos(counter(1), counter(2), counter(3), counter(4), counter(5), counter(6), counter(7));}
  (junction 3189) -> (junction 3214) : {timer_spuren = countOnwards(timer_spuren,3,[1 1 1 1 1 0 1]);}
  (junction 1185) -> (junction 1180) : {wartezeiten2 = berechne_wartezeiten(startzeiten2, endzeiten2, alte_counter(2), counter(2), wartezeiten2);}
  (junction 3551) -> (junction 3561) : {wartezeiten6 = berechne_wartezeiten(startzeiten6, endzeiten6, alte_counter(6), counter(6), wartezeiten6);}
  (junction 3169) -> (junction 3209) : {timer_spuren = countOnwards(timer_spuren,1,[1 1 1 1 1 0 0]);}
  rg3_fuss5_rot8 -> (junction 3562) : {[anz_autos6, autos_auf_spur6, counter(6), endzeiten6] = generiere_gruenphase(6, 12, autos_auf_spur6, counter(6),  (gesamtZeit + timeCounter - 12), endzeiten6, startzeiten6, auslastung, autos_spur1_flag);}
  (junction 3214) -> rg3_rot_ampel4_rotgelb6 : {[autos_auf_spur6, spur6] = autos_auf_spur_generieren(spur6, gesamtZeit + timeCounter, autos_auf_spur6);}
  (junction 1180) -> (junction 1175) : {wartezeit_spur2_ges = gesamt_wartezeit_pro_spur(wartezeiten2, wartezeit_spur2_ges, alte_counter(2), counter(2));}
  (junction 3561) -> (junction 3579) : {wartezeit_spur6_ges = gesamt_wartezeit_pro_spur(wartezeiten6, wartezeit_spur6_ges, alte_counter(6), counter(6));}
  (junction 1826) -> (junction 1824) : {wartezeiten6 = berechne_wartezeiten(startzeiten6, endzeiten6, alte_counter(6), counter(6), wartezeiten6);}
  rg3_rot_ampel4_rotgelb1 -> (junction 1187) : after(1,sec)
      | {timeCounter = refresher(timeCounter, 1);}
  rg3_fuss5_rot2 -> (junction 1829) : {[anz_autos6, autos_auf_spur6, counter(6), endzeiten6] = generiere_gruenphase(6, 17, autos_auf_spur6, counter(6),  (gesamtZeit + timeCounter -17), endzeiten6, startzeiten6, auslastung, autos_spur1_flag);}
  (junction 1824) -> (junction 1825) : {wartezeit_spur6_ges = gesamt_wartezeit_pro_spur(wartezeiten6, wartezeit_spur6_ges, alte_counter(6), counter(6));}
  (junction 1175) -> (junction 1195) : {gesamtwartezeit = berechne_gesamtwartezeit(wartezeit_spur1_ges, wartezeit_spur2_ges, wartezeit_spur3_ges, wartezeit_spur4_ges, wartezeit_spur5_ges, wartezeit_spur6_ges, wartezeit_spur7_ges);}
  (junction 3579) -> (junction 3573) : {gesamtwartezeit = berechne_gesamtwartezeit(wartezeit_spur1_ges, wartezeit_spur2_ges, wartezeit_spur3_ges, wartezeit_spur4_ges, wartezeit_spur5_ges, wartezeit_spur6_ges, wartezeit_spur7_ges);}
  (junction 3209) -> rg3_fuss5_rot6 : {[autos_auf_spur6, spur6] = autos_auf_spur_generieren(spur6, gesamtZeit + timeCounter, autos_auf_spur6);}
  (junction 1187) -> ampel4_fuss5_gruen1 : {timer_spuren = countOnwards(timer_spuren,1,[1 1 1 1 1 1 1]);}
  rg3_rot_ampel4_rotgelb6 -> (junction 3204) : {[anz_autos6, autos_auf_spur6, counter(6), endzeiten6] = generiere_gruenphase(6, 10, autos_auf_spur6, counter(6),  (gesamtZeit + timeCounter - 10), endzeiten6, startzeiten6, auslastung, autos_spur1_flag);}
  (junction 1195) -> rg3_fuss5_rot1 : {gesamte_autos = berechne_gesamte_autos(counter(1), counter(2), counter(3), counter(4), counter(5), counter(6), counter(7));}
  (junction 3573) -> rg3_rot_ampel4_rotgelb9 : {gesamte_autos = berechne_gesamte_autos(counter(1), counter(2), counter(3), counter(4), counter(5), counter(6), counter(7));}
  (junction 1825) -> (junction 1807) : {gesamtwartezeit = berechne_gesamtwartezeit(wartezeit_spur1_ges, wartezeit_spur2_ges, wartezeit_spur3_ges, wartezeit_spur4_ges, wartezeit_spur5_ges, wartezeit_spur6_ges, wartezeit_spur7_ges);}
  (junction 3562) -> (junction 3571) : {wartezeiten2 = berechne_wartezeiten(startzeiten2, endzeiten2, alte_counter(2), counter(2), wartezeiten2);}
  (junction 1807) -> rg3_rot_ampel4_rotgelb3 : {gesamte_autos = berechne_gesamte_autos(counter(1), counter(2), counter(3), counter(4), counter(5), counter(6), counter(7));}
  (junction 3571) -> (junction 3564) : {wartezeit_spur2_ges = gesamt_wartezeit_pro_spur(wartezeiten2, wartezeit_spur2_ges, alte_counter(2), counter(2));}
  (junction 1829) -> (junction 1828) : {wartezeiten2 = berechne_wartezeiten(startzeiten2, endzeiten2, alte_counter(2), counter(2), wartezeiten2);}
  (junction 3204) -> (junction 3205) : {wartezeiten6 = berechne_wartezeiten(startzeiten6, endzeiten6, alte_counter(6), counter(6), wartezeiten6);}
  rg3_rot_ampel4_rotgelb9 -> (junction 3559) : after(1,sec)
      | {timeCounter = refresher(timeCounter, 1);}
  ampel4_fuss5_gruen1 -> (junction 1167) : {[autos_auf_spur7, spur7] = autos_auf_spur_generieren(spur7, gesamtZeit + timeCounter, autos_auf_spur7);}
  rg3_fuss5_rot6 -> (junction 3220) : {[anz_autos6, autos_auf_spur6, counter(6), endzeiten6] = generiere_gruenphase(6, 10, autos_auf_spur6, counter(6),  (gesamtZeit + timeCounter -10), endzeiten6, startzeiten6, auslastung, autos_spur1_flag);}
  (junction 1828) -> (junction 1816) : {wartezeit_spur2_ges = gesamt_wartezeit_pro_spur(wartezeiten2, wartezeit_spur2_ges, alte_counter(2), counter(2));}
  (junction 1167) -> (junction 1170) : after(11,sec)
      | {timeCounter = refresher(timeCounter, 11);}
  (junction 3564) -> (junction 3557) : {gesamtwartezeit = berechne_gesamtwartezeit(wartezeit_spur1_ges, wartezeit_spur2_ges, wartezeit_spur3_ges, wartezeit_spur4_ges, wartezeit_spur5_ges, wartezeit_spur6_ges, wartezeit_spur7_ges);}
  (junction 3205) -> (junction 3217) : {wartezeit_spur6_ges = gesamt_wartezeit_pro_spur(wartezeiten6, wartezeit_spur6_ges, alte_counter(6), counter(6));}
  rg3_rot_ampel4_rotgelb3 -> (junction 1808) : after(1,sec)
      | {timeCounter = refresher(timeCounter, 1);}
  (junction 3559) -> ampel4_fuss5_gruen9 : {timer_spuren = countOnwards(timer_spuren,1,[1 1 1 1 1 1 1]);}
  (junction 3557) -> rg3_fuss5_rot9 : {gesamte_autos = berechne_gesamte_autos(counter(1), counter(2), counter(3), counter(4), counter(5), counter(6), counter(7));}
  (junction 1816) -> (junction 1811) : {gesamtwartezeit = berechne_gesamtwartezeit(wartezeit_spur1_ges, wartezeit_spur2_ges, wartezeit_spur3_ges, wartezeit_spur4_ges, wartezeit_spur5_ges, wartezeit_spur6_ges, wartezeit_spur7_ges);}
  (junction 1170) -> fuss5_rot : {timer_spuren = countOnwards(timer_spuren,11,[1 1 1 1 1 1 0]);}
  (junction 3217) -> (junction 3212) : {gesamtwartezeit = berechne_gesamtwartezeit(wartezeit_spur1_ges, wartezeit_spur2_ges, wartezeit_spur3_ges, wartezeit_spur4_ges, wartezeit_spur5_ges, wartezeit_spur6_ges, wartezeit_spur7_ges);}
  (junction 1808) -> ampel4_fuss5_gruen3 : {timer_spuren = countOnwards(timer_spuren,1,[1 1 1 1 1 1 1]);}
  (junction 1811) -> rg3_fuss5_rot3 : {gesamte_autos = berechne_gesamte_autos(counter(1), counter(2), counter(3), counter(4), counter(5), counter(6), counter(7));}
  (junction 3212) -> rg3_rot_ampel4_rotgelb7 : {gesamte_autos = berechne_gesamte_autos(counter(1), counter(2), counter(3), counter(4), counter(5), counter(6), counter(7));}
  fuss5_rot -> (junction 1165)
  (junction 3220) -> (junction 3206) : {wartezeiten2 = berechne_wartezeiten(startzeiten2, endzeiten2, alte_counter(2), counter(2), wartezeiten2);}
  ampel4_fuss5_gruen9 -> (junction 3569) : {[autos_auf_spur7, spur7] = autos_auf_spur_generieren(spur7, gesamtZeit + timeCounter, autos_auf_spur7);}
  (junction 3569) -> (junction 3581) : after(7,sec)
      | {timeCounter = refresher(timeCounter, 7);}
  (junction 3206) -> (junction 3215) : {wartezeit_spur2_ges = gesamt_wartezeit_pro_spur(wartezeiten2, wartezeit_spur2_ges, alte_counter(2), counter(2));}
  ampel4_fuss5_gruen3 -> (junction 1803) : {[autos_auf_spur7, spur7] = autos_auf_spur_generieren(spur7, gesamtZeit + timeCounter, autos_auf_spur7);}
  rg3_rot_ampel4_rotgelb7 -> (junction 3207) : after(1,sec)
      | {timeCounter = refresher(timeCounter, 1);}
  (junction 1803) -> (junction 1802) : after(11,sec)
      | {timeCounter = refresher(timeCounter, 11);}
  (junction 3581) -> fuss5_rot4 : {timer_spuren = countOnwards(timer_spuren,7,[1 1 1 1 1 1 0]);}
  (junction 3215) -> (junction 3198) : {gesamtwartezeit = berechne_gesamtwartezeit(wartezeit_spur1_ges, wartezeit_spur2_ges, wartezeit_spur3_ges, wartezeit_spur4_ges, wartezeit_spur5_ges, wartezeit_spur6_ges, wartezeit_spur7_ges);}
  rg3_fuss5_rot1 -> (junction 1168)
  (junction 3207) -> ampel4_fuss5_gruen7 : {timer_spuren = countOnwards(timer_spuren,1,[1 1 1 1 1 1 1]);}
  (junction 3198) -> rg3_fuss5_rot7 : {gesamte_autos = berechne_gesamte_autos(counter(1), counter(2), counter(3), counter(4), counter(5), counter(6), counter(7));}
  (junction 1802) -> fuss5_rot1 : {timer_spuren = countOnwards(timer_spuren,11,[1 1 1 1 1 1 0]);}
  fuss5_rot4 -> (junction 3574)
  fuss5_rot1 -> (junction 1820)
  ampel4_fuss5_gruen7 -> (junction 3208) : {[autos_auf_spur7, spur7] = autos_auf_spur_generieren(spur7, gesamtZeit + timeCounter, autos_auf_spur7);}
  (junction 1165) -> (junction 1184)
  (junction 1168) -> (junction 1165)
  (junction 3208) -> (junction 3222) : after(3,sec)
      | {timeCounter = refresher(timeCounter, 3);}
  (junction 1184) -> (junction 1173) : after(2,sec)
      | {timeCounter = refresher(timeCounter, 2);}
  rg3_fuss5_rot9 -> (junction 3554)
  (junction 3222) -> fuss5_rot3 : {timer_spuren = countOnwards(timer_spuren,3,[1 1 1 1 1 1 0]);}
  rg3_fuss5_rot3 -> (junction 1801)
  (junction 1173) -> ampel4_gelb : {timer_spuren = countOnwards(timer_spuren,2,[1 1 1 1 1 1 0]);}
  fuss5_rot3 -> (junction 3194) : after(2,sec)
      | {timeCounter = refresher(timeCounter, 2);}
  (junction 3574) -> (junction 3563)
  (junction 3554) -> (junction 3574)
  (junction 3563) -> (junction 3575) : %after(1,sec)
      | %{timeCounter = refresher(timeCounter, 1);}
  ampel4_gelb -> (junction 1174) : after(3,sec)
      | {timeCounter = refresher(timeCounter, 3);}
  (junction 1174) -> (junction 1178) : {timer_spuren = countOnwards(timer_spuren,3,[1 1 1 1 1 1 0]);}
  (junction 1820) -> (junction 1800)
  (junction 1801) -> (junction 1820)
  (junction 1800) -> (junction 1804) : after(2,sec)
      | {timeCounter = refresher(timeCounter, 2);}
  (junction 1178) -> ampel4_rot : {[autos_auf_spur7, spur7] = autos_auf_spur_generieren(spur7, gesamtZeit + timeCounter, autos_auf_spur7);}
  rg3_fuss5_rot7 -> (junction 3221) : after(2,sec)
      | {timeCounter = refresher(timeCounter, 2);}
  (junction 3575) -> ampel4_gelb4 : %{timer_spuren = countOnwards(timer_spuren,1,[1 1 1 1 1 1 0]);}
  (junction 3194) -> (junction 3210) : {timer_spuren = countOnwards(timer_spuren,2,[1 1 1 1 1 1 0]);}
  ampel4_rot -> ampel4_rot2 : {[anz_autos7, autos_auf_spur7, counter(7), endzeiten7] = generiere_gruenphase(7, 16, autos_auf_spur7, counter(7),  (gesamtZeit + timeCounter -16), endzeiten7, startzeiten7, auslastung, autos_spur1_flag);}
  (junction 1804) -> ampel4_gelb1 : {timer_spuren = countOnwards(timer_spuren,2,[1 1 1 1 1 1 0]);}
  (junction 3221) -> (junction 3216) : {timer_spuren = countOnwards(timer_spuren,2,[1 1 1 1 1 1 0]);}
  ampel4_gelb4 -> (junction 3576) : after(3,sec)
      | {timeCounter = refresher(timeCounter, 3);}
  ampel4_rot2 -> (junction 1181) : after(4,sec)
      | {timeCounter = refresher(timeCounter, 4);}
  (junction 3576) -> (junction 3577) : {timer_spuren = countOnwards(timer_spuren,3,[1 1 1 1 1 1 0]);}
  (junction 3210) -> (junction 3203)
  (junction 3216) -> (junction 3210)
  (junction 3203) -> ampel4_gelb3
  ampel4_gelb1 -> (junction 1809) : after(3,sec)
      | {timeCounter = refresher(timeCounter, 3);}
  (junction 3577) -> ampel4_rot9 : {[autos_auf_spur7, spur7] = autos_auf_spur_generieren(spur7, gesamtZeit + timeCounter, autos_auf_spur7);}
  (junction 1181) -> (junction 1183) : {timer_spuren = countOnwards(timer_spuren,4,[1 1 1 1 1 1 1]);}
  (junction 1809) -> (junction 1805) : {timer_spuren = countOnwards(timer_spuren,3,[1 1 1 1 1 1 0]);}
  (junction 1183) -> (junction 1205) : {gesamtZeit = gesamtZeit + timeCounter;}
  (junction 1205) -> (junction 1207) : %{disp(startzeiten1)}
  (junction 1805) -> ampel4_rot3 : {[autos_auf_spur7, spur7] = autos_auf_spur_generieren(spur7, gesamtZeit + timeCounter, autos_auf_spur7);}
  ampel4_rot9 -> ampel4_rot10 : {[anz_autos7, autos_auf_spur7, counter(7), endzeiten7] = generiere_gruenphase(7, 10, autos_auf_spur7, counter(7),  (gesamtZeit + timeCounter - 10), endzeiten7, startzeiten7, auslastung, autos_spur1_flag);}
  (junction 1207) -> (junction 1215) : %{disp(endzeiten1)}
  (junction 1215) -> (junction 1212) : {wartezeiten1 = berechne_wartezeiten(startzeiten1, endzeiten1, alte_counter(1), counter(1), wartezeiten1);}
  ampel4_rot3 -> ampel4_rot4 : {[anz_autos7, autos_auf_spur7, counter(7), endzeiten7] = generiere_gruenphase(7, 16, autos_auf_spur7, counter(7),  (gesamtZeit + timeCounter -16), endzeiten7, startzeiten7, auslastung, autos_spur1_flag);}
  (junction 1212) -> (junction 1223) : {wartezeit_spur1_ges = gesamt_wartezeit_pro_spur(wartezeiten1, wartezeit_spur1_ges, alte_counter(1), counter(1));}
  ampel4_rot10 -> (junction 3578) : after(4,sec)
      | {timeCounter = refresher(timeCounter, 4);}
  (junction 1223) -> (junction 1214) : {wartezeiten2 = berechne_wartezeiten(startzeiten2, endzeiten2, alte_counter(2), counter(2), wartezeiten2);}
  ampel4_gelb3 -> (junction 3211) : after(3,sec)
      | {timeCounter = refresher(timeCounter, 3);}
  (junction 3578) -> (junction 3555) : {timer_spuren = countOnwards(timer_spuren,4,[1 1 1 1 1 1 1]);}
  ampel4_rot4 -> (junction 1831) : after(4,sec)
      | {timeCounter = refresher(timeCounter, 4);}
  (junction 3555) -> (junction 3556) : {gesamtZeit = gesamtZeit + timeCounter;}
  (junction 3211) -> (junction 3199) : {timer_spuren = countOnwards(timer_spuren,3,[1 1 1 1 1 1 0]);}
  (junction 1214) -> (junction 1198) : {wartezeit_spur2_ges = gesamt_wartezeit_pro_spur(wartezeiten2, wartezeit_spur2_ges, alte_counter(2), counter(2));}
  (junction 3556) -> (junction 3566) : %{disp(startzeiten1)}
  (junction 1831) -> (junction 1817) : {timer_spuren = countOnwards(timer_spuren,4,[1 1 1 1 1 1 1]);}
  (junction 3199) -> ampel4_rot7 : {[autos_auf_spur7, spur7] = autos_auf_spur_generieren(spur7, gesamtZeit + timeCounter, autos_auf_spur7);}
  (junction 3566) -> (junction 3565) : %{disp(endzeiten1)}
  (junction 1817) -> (junction 1806) : {gesamtZeit = gesamtZeit + timeCounter;}
  (junction 1198) -> (junction 1222) : {wartezeiten3 = berechne_wartezeiten(startzeiten3, endzeiten3, alte_counter(3), counter(3), wartezeiten3);}
  (junction 3565) -> (junction 3567) : {wartezeiten1 = berechne_wartezeiten(startzeiten1, endzeiten1, alte_counter(1), counter(1), wartezeiten1);}
  (junction 1806) -> (junction 1810) : %{disp(startzeiten1)}
  ampel4_rot7 -> ampel4_rot8 : {[anz_autos7, autos_auf_spur7, counter(7), endzeiten7] = generiere_gruenphase(7, 10, autos_auf_spur7, counter(7),  (gesamtZeit + timeCounter -10), endzeiten7, startzeiten7, auslastung, autos_spur1_flag);}
  (junction 1810) -> (junction 1812) : %{disp(endzeiten1)}
  (junction 3567) -> (junction 3558) : {wartezeit_spur1_ges = gesamt_wartezeit_pro_spur(wartezeiten1, wartezeit_spur1_ges, alte_counter(1), counter(1));}
  (junction 1222) -> (junction 1209) : {wartezeit_spur3_ges = gesamt_wartezeit_pro_spur(wartezeiten3, wartezeit_spur3_ges, alte_counter(3), counter(3));}
  (junction 1812) -> (junction 1814) : {wartezeiten1 = berechne_wartezeiten(startzeiten1, endzeiten1, alte_counter(1), counter(1), wartezeiten1);}
  (junction 3558) -> (junction 3568) : {wartezeiten2 = berechne_wartezeiten(startzeiten2, endzeiten2, alte_counter(2), counter(2), wartezeiten2);}
  (junction 1209) -> (junction 1206) : {wartezeiten4 = berechne_wartezeiten(startzeiten4, endzeiten4, alte_counter(4), counter(4), wartezeiten4);}
  (junction 1814) -> (junction 1827) : {wartezeit_spur1_ges = gesamt_wartezeit_pro_spur(wartezeiten1, wartezeit_spur1_ges, alte_counter(1), counter(1));}
  ampel4_rot8 -> (junction 3193) : after(4,sec)
      | {timeCounter = refresher(timeCounter, 4);}
  (junction 3568) -> (junction 3572) : {wartezeit_spur2_ges = gesamt_wartezeit_pro_spur(wartezeiten2, wartezeit_spur2_ges, alte_counter(2), counter(2));}
  (junction 1206) -> (junction 1213) : {wartezeit_spur4_ges = gesamt_wartezeit_pro_spur(wartezeiten4, wartezeit_spur4_ges, alte_counter(4), counter(4));}
  (junction 1827) -> (junction 1813) : {wartezeiten2 = berechne_wartezeiten(startzeiten2, endzeiten2, alte_counter(2), counter(2), wartezeiten2);}
  (junction 3193) -> (junction 3201) : {timer_spuren = countOnwards(timer_spuren,4,[1 1 1 1 1 1 1]);}
  (junction 1213) -> (junction 1200) : {wartezeiten5 = berechne_wartezeiten(startzeiten5, endzeiten5, alte_counter(5), counter(5), wartezeiten5);}
  (junction 3201) -> (junction 3218) : {gesamtZeit = gesamtZeit + timeCounter;}
  (junction 3572) -> (junction 3580) : {wartezeiten3 = berechne_wartezeiten(startzeiten3, endzeiten3, alte_counter(3), counter(3), wartezeiten3);}
  (junction 1813) -> (junction 1815) : {wartezeit_spur2_ges = gesamt_wartezeit_pro_spur(wartezeiten2, wartezeit_spur2_ges, alte_counter(2), counter(2));}
  (junction 1200) -> (junction 1220) : {wartezeit_spur5_ges = gesamt_wartezeit_pro_spur(wartezeiten5, wartezeit_spur5_ges, alte_counter(5), counter(5));}
  (junction 3218) -> (junction 3191) : %{disp(startzeiten1)}
  (junction 3191) -> (junction 3213) : %{disp(endzeiten1)}
  (junction 1220) -> (junction 1219) : {wartezeiten6 = berechne_wartezeiten(startzeiten6, endzeiten6, alte_counter(6), counter(6), wartezeiten6);}
  (junction 3580) -> (junction 3582) : {wartezeit_spur3_ges = gesamt_wartezeit_pro_spur(wartezeiten3, wartezeit_spur3_ges, alte_counter(3), counter(3));}
  (junction 1815) -> (junction 1818) : {wartezeiten3 = berechne_wartezeiten(startzeiten3, endzeiten3, alte_counter(3), counter(3), wartezeiten3);}
  (junction 3213) -> (junction 3196) : {wartezeiten1 = berechne_wartezeiten(startzeiten1, endzeiten1, alte_counter(1), counter(1), wartezeiten1);}
  (junction 1219) -> (junction 1217) : {wartezeit_spur6_ges = gesamt_wartezeit_pro_spur(wartezeiten6, wartezeit_spur6_ges, alte_counter(6), counter(6));}
  (junction 3582) -> (junction 3560) : {wartezeiten4 = berechne_wartezeiten(startzeiten4, endzeiten4, alte_counter(4), counter(4), wartezeiten4);}
  (junction 1818) -> (junction 1830) : {wartezeit_spur3_ges = gesamt_wartezeit_pro_spur(wartezeiten3, wartezeit_spur3_ges, alte_counter(3), counter(3));}
  (junction 3196) -> (junction 3192) : {wartezeit_spur1_ges = gesamt_wartezeit_pro_spur(wartezeiten1, wartezeit_spur1_ges, alte_counter(1), counter(1));}
  (junction 1217) -> (junction 1216) : %{disp(startzeiten7)}
  (junction 3560) -> (junction 3583) : {wartezeit_spur4_ges = gesamt_wartezeit_pro_spur(wartezeiten4, wartezeit_spur4_ges, alte_counter(4), counter(4));}
  (junction 3192) -> (junction 3200) : {wartezeiten2 = berechne_wartezeiten(startzeiten2, endzeiten2, alte_counter(2), counter(2), wartezeiten2);}
  (junction 1830) -> (junction 1819) : {wartezeiten4 = berechne_wartezeiten(startzeiten4, endzeiten4, alte_counter(4), counter(4), wartezeiten4);}
  (junction 3583) -> (junction 3584) : {wartezeiten5 = berechne_wartezeiten(startzeiten5, endzeiten5, alte_counter(5), counter(5), wartezeiten5);}
  (junction 1216) -> (junction 1208) : %{disp(endzeiten7)}
  (junction 3200) -> (junction 3219) : {wartezeit_spur2_ges = gesamt_wartezeit_pro_spur(wartezeiten2, wartezeit_spur2_ges, alte_counter(2), counter(2));}
  (junction 1819) -> (junction 1821) : {wartezeit_spur4_ges = gesamt_wartezeit_pro_spur(wartezeiten4, wartezeit_spur4_ges, alte_counter(4), counter(4));}
  (junction 3584) -> (junction 3570) : {wartezeit_spur5_ges = gesamt_wartezeit_pro_spur(wartezeiten5, wartezeit_spur5_ges, alte_counter(5), counter(5));}
  (junction 1821) -> (junction 1822) : {wartezeiten5 = berechne_wartezeiten(startzeiten5, endzeiten5, alte_counter(5), counter(5), wartezeiten5);}
  (junction 3570) -> (junction 3553) : {wartezeiten6 = berechne_wartezeiten(startzeiten6, endzeiten6, alte_counter(6), counter(6), wartezeiten6);}
  (junction 1208) -> (junction 1199) : {wartezeiten7 = berechne_wartezeiten(startzeiten7, endzeiten7, alte_counter(7), counter(7), wartezeiten7);}
  (junction 3219) -> (junction 3195) : {wartezeiten3 = berechne_wartezeiten(startzeiten3, endzeiten3, alte_counter(3), counter(3), wartezeiten3);}
  (junction 1822) -> (junction 1823) : {wartezeit_spur5_ges = gesamt_wartezeit_pro_spur(wartezeiten5, wartezeit_spur5_ges, alte_counter(5), counter(5));}
  (junction 3553) -> (junction 3588) : {wartezeit_spur6_ges = gesamt_wartezeit_pro_spur(wartezeiten6, wartezeit_spur6_ges, alte_counter(6), counter(6));}
  (junction 1823) -> (junction 1832) : {wartezeiten6 = berechne_wartezeiten(startzeiten6, endzeiten6, alte_counter(6), counter(6), wartezeiten6);}
  (junction 3195) -> (junction 3197) : {wartezeit_spur3_ges = gesamt_wartezeit_pro_spur(wartezeiten3, wartezeit_spur3_ges, alte_counter(3), counter(3));}
  (junction 1199) -> (junction 1196) : {wartezeit_spur7_ges = gesamt_wartezeit_pro_spur(wartezeiten7, wartezeit_spur7_ges, alte_counter(7), counter(7));}
  (junction 3588) -> (junction 3611) : %{disp(startzeiten7)}
  (junction 1832) -> (junction 1837) : {wartezeit_spur6_ges = gesamt_wartezeit_pro_spur(wartezeiten6, wartezeit_spur6_ges, alte_counter(6), counter(6));}
  (junction 3197) -> (junction 3202) : {wartezeiten4 = berechne_wartezeiten(startzeiten4, endzeiten4, alte_counter(4), counter(4), wartezeiten4);}
  (junction 3611) -> (junction 3613) : %{disp(endzeiten7)}
  (junction 1837) -> (junction 1833) : %{disp(startzeiten7)}
  (junction 3202) -> (junction 3235) : {wartezeit_spur4_ges = gesamt_wartezeit_pro_spur(wartezeiten4, wartezeit_spur4_ges, alte_counter(4), counter(4));}
  (junction 1196) -> (junction 1218) : {gesamtwartezeit = berechne_gesamtwartezeit(wartezeit_spur1_ges, wartezeit_spur2_ges, wartezeit_spur3_ges, wartezeit_spur4_ges, wartezeit_spur5_ges, wartezeit_spur6_ges, wartezeit_spur7_ges)}
  (junction 1833) -> (junction 1835) : %{disp(endzeiten7)}
  (junction 3613) -> (junction 3609) : {wartezeiten7 = berechne_wartezeiten(startzeiten7, endzeiten7, alte_counter(7), counter(7), wartezeiten7);}
  (junction 3235) -> (junction 3229) : {wartezeiten5 = berechne_wartezeiten(startzeiten5, endzeiten5, alte_counter(5), counter(5), wartezeiten5);}
  (junction 3229) -> (junction 3232) : {wartezeit_spur5_ges = gesamt_wartezeit_pro_spur(wartezeiten5, wartezeit_spur5_ges, alte_counter(5), counter(5));}
  (junction 1835) -> (junction 1838) : {wartezeiten7 = berechne_wartezeiten(startzeiten7, endzeiten7, alte_counter(7), counter(7), wartezeiten7);}
  (junction 3232) -> (junction 3234) : {wartezeiten6 = berechne_wartezeiten(startzeiten6, endzeiten6, alte_counter(6), counter(6), wartezeiten6);}
  (junction 3609) -> (junction 3604) : {wartezeit_spur7_ges = gesamt_wartezeit_pro_spur(wartezeiten7, wartezeit_spur7_ges, alte_counter(7), counter(7));}
  (junction 1218) -> (junction 1201) : {gesamte_autos = berechne_gesamte_autos(counter(1), counter(2), counter(3), counter(4), counter(5), counter(6), counter(7))}
  (junction 3234) -> (junction 3223) : {wartezeit_spur6_ges = gesamt_wartezeit_pro_spur(wartezeiten6, wartezeit_spur6_ges, alte_counter(6), counter(6));}
  (junction 1838) -> (junction 1834) : {wartezeit_spur7_ges = gesamt_wartezeit_pro_spur(wartezeiten7, wartezeit_spur7_ges, alte_counter(7), counter(7));}
  (junction 3223) -> (junction 3230) : %{disp(startzeiten7)}
  (junction 1201) -> (junction 1202) : {runden_ueberquerte_autos = counter(1) - alte_counter(1) + counter(2) - alte_counter(2) + counter(3) - alte_counter(3) + counter(4) - alte_counter(4) + counter(5) - alte_counter(5) + counter(6) - alte_counter(6) + counter(7) - alte_counter(7);}
  (junction 3604) -> (junction 3599) : {gesamtwartezeit = berechne_gesamtwartezeit(wartezeit_spur1_ges, wartezeit_spur2_ges, wartezeit_spur3_ges, wartezeit_spur4_ges, wartezeit_spur5_ges, wartezeit_spur6_ges, wartezeit_spur7_ges)}
  (junction 3230) -> (junction 3227) : %{disp(endzeiten7)}
  (junction 1202) -> (junction 1221) : {krit1 = runden_ueberquerte_autos / timeCounter;}
  (junction 1834) -> (junction 1836) : {gesamtwartezeit = berechne_gesamtwartezeit(wartezeit_spur1_ges, wartezeit_spur2_ges, wartezeit_spur3_ges, wartezeit_spur4_ges, wartezeit_spur5_ges, wartezeit_spur6_ges, wartezeit_spur7_ges)}
  (junction 3227) -> (junction 3224) : {wartezeiten7 = berechne_wartezeiten(startzeiten7, endzeiten7, alte_counter(7), counter(7), wartezeiten7);}
  (junction 3599) -> (junction 3614) : {gesamte_autos = berechne_gesamte_autos(counter(1), counter(2), counter(3), counter(4), counter(5), counter(6), counter(7))}
  (junction 1221) -> (junction 1203) : {krit2 = gesamte_autos / (gesamtZeit + timeCounter);}
  (junction 3224) -> (junction 3233) : {wartezeit_spur7_ges = gesamt_wartezeit_pro_spur(wartezeiten7, wartezeit_spur7_ges, alte_counter(7), counter(7));}
  (junction 1836) -> (junction 1441) : {gesamte_autos = berechne_gesamte_autos(counter(1), counter(2), counter(3), counter(4), counter(5), counter(6), counter(7))}
  (junction 3614) -> (junction 3603) : {runden_ueberquerte_autos = counter(1) - alte_counter(1) + counter(2) - alte_counter(2) + counter(3) - alte_counter(3) + counter(4) - alte_counter(4) + counter(5) - alte_counter(5) + counter(6) - alte_counter(6) + counter(7) - alte_counter(7);}
  (junction 1203) -> (junction 1204) : {krit3 = gesamtwartezeit / gesamte_autos;}
  (junction 1441) -> (junction 1437) : {runden_ueberquerte_autos = counter(1) - alte_counter(1) + counter(2) - alte_counter(2) + counter(3) - alte_counter(3) + counter(4) - alte_counter(4) + counter(5) - alte_counter(5) + counter(6) - alte_counter(6) + counter(7) - alte_counter(7);}
  (junction 3603) -> (junction 3619) : {krit1 = runden_ueberquerte_autos / timeCounter;}
  (junction 3233) -> (junction 3226) : {gesamtwartezeit = berechne_gesamtwartezeit(wartezeit_spur1_ges, wartezeit_spur2_ges, wartezeit_spur3_ges, wartezeit_spur4_ges, wartezeit_spur5_ges, wartezeit_spur6_ges, wartezeit_spur7_ges)}
  (junction 1437) -> (junction 1433) : {krit1 = runden_ueberquerte_autos / timeCounter;}
  (junction 1204) -> (junction 3349)
  (junction 3619) -> (junction 3622) : {krit2 = gesamte_autos / (gesamtZeit + timeCounter);}
  (junction 3226) -> (junction 3231) : {gesamte_autos = berechne_gesamte_autos(counter(1), counter(2), counter(3), counter(4), counter(5), counter(6), counter(7))}
  (junction 1433) -> (junction 1434) : {krit2 = gesamte_autos / (gesamtZeit + timeCounter);}
  (junction 3622) -> (junction 3595) : {krit3 = gesamtwartezeit / gesamte_autos;}
  (junction 3231) -> (junction 3237) : {runden_ueberquerte_autos = counter(1) - alte_counter(1) + counter(2) - alte_counter(2) + counter(3) - alte_counter(3) + counter(4) - alte_counter(4) + counter(5) - alte_counter(5) + counter(6) - alte_counter(6) + counter(7) - alte_counter(7);}
  (junction 3595) -> (junction 3343)
  (junction 1434) -> (junction 1478) : {krit3 = gesamtwartezeit / gesamte_autos;}
  (junction 3237) -> (junction 3236) : {krit1 = runden_ueberquerte_autos / timeCounter;}
  (junction 1478) -> (junction 3346)
  (junction 3236) -> (junction 3225) : {krit2 = gesamte_autos / (gesamtZeit + timeCounter);}
  (junction 3225) -> (junction 3228) : {krit3 = gesamtwartezeit / gesamte_autos;}
  (junction 3228) -> (junction 3338)
  (junction 3338) -> (junction 179)
  (junction 3343) -> (junction 3338)
  (junction 3346) -> (junction 3343)
  (junction 3349) -> (junction 3346)
  data: autos_neu_fkt function_output; N_fkt function_input; zeit_abstand_fkt function_input; auslastung_fkt function_input; autos_fkt function_input; spur1fkt function_output; spur2fkt function_output; spur3fkt function_output; spur4fkt function_output; spur5fkt function_output; spur6fkt function_output; spur7fkt function_output; N_fkt function_input; spur_autos function_input; timer function_input; autos_auf_spur_fkt function_input; autos_auf_spur_fkt function_output; spur_autos function_output; spur function_input; laenge function_input; autos_auf_spur_u function_input; counter_alt function_input; start_timer_fkt function_input; endzeiten function_input; anz_autos_fkt function_output; autos_auf_spur_fkt function_output; counter_neu_fkt function_output; endzeiten function_output; startzeiten_fkt function_input; auslastung_fkt function_input; autos_spur1_flag_fkt function_input; auslastung_fkt function_input; zeit_abstand_fkt function_output; time function_input; timeElapsed function_input; spuren function_input; count_spur function_output; timer function_output; timer function_output; startTime function_input; timeElapsed function_input; startzeiten_fkt function_input; endzeiten_fkt function_input; alter_counter_fkt function_input; counter_fkt function_input; wartezeiten_fkt_u function_input; wartezeiten_fkt function_output; wartezeit_fkt function_input; spur_wartezeit_u function_input; counter_alt_fkt function_input; spur_wartezeit_fkt function_output double; counter_fkt function_input; ges_wartezeit1_fkt function_input; ges_wartezeit2_fkt function_input; ges_wartezeit3_fkt function_input; ges_wartezeit4_fkt function_input; ges_wartezeit5_fkt function_input; ges_wartezeit6_fkt function_input; ges_wartezeit7_fkt function_input; gesamtwartezeit_fkt function_output; counter1_fkt function_input; counter2_fkt function_input; counter3_fkt function_input; counter4_fkt function_input; counter5_fkt function_input; counter6_fkt function_input; counter7_fkt function_input; gesamte_autos_fkt function_output; rot1_l output; gelb1_l output; gruen1_l output; rot1_rg output; gelb1_rg output; gruen1_rg output; rot2 output; gelb2 output; gruen2 output; rot3_l output; gelb3_l output; gruen3_l output; rot3_rg output; gelb3_rg output; gruen3_rg output; rot4 output; gelb4 output; gruen4 output; rot5 output; gruen5 output; rot6 output; gruen6 output; rot7 output; gruen7 output; rot8 output; gruen8 output; autos_auf_spur1 output; timer_spuren local; anz_autos1 local; anz_autos2 local; anz_autos3 local; anz_autos4 local; anz_autos5 local; anz_autos6 local; anz_autos7 local; alte_counter local; counter local; endzeiten1 local; endzeiten2 local; endzeiten3 local; endzeiten4 local; endzeiten5 local; endzeiten6 local; endzeiten7 local; spur1 local; spur2 local; spur3 local; spur4 local; spur5 local; spur6 local; spur7 local; startzeiten7 local; wartezeiten1 local; startzeiten1 local; startzeiten2 local; startzeiten3 local; startzeiten4 local; startzeiten5 local; startzeiten6 local; wartezeiten2 local; wartezeiten3 local; wartezeiten4 local; wartezeiten5 local; wartezeiten6 local; wartezeiten7 local; autos_auf_spur2 output; autos_auf_spur3 output; autos_auf_spur4 output; autos_auf_spur5 output; autos_auf_spur6 output; autos_auf_spur7 output; wartezeit_spur1_ges output; wartezeit_spur2_ges output; wartezeit_spur3_ges output; wartezeit_spur4_ges output; wartezeit_spur5_ges output; wartezeit_spur6_ges output; wartezeit_spur7_ges output; gesamtwartezeit output; timeCounter output; gesamtZeit output; alle_autos_neu local; N constant double =10000; auslastung input; zeit_abstand local; gesamte_autos output; krit1 output; krit2 output; runden_ueberquerte_autos local; krit3 output; autos_spur1_flag local
  function autos_neu_fkt = generiere_autos_neu(N_fkt, zeit_abstand_fkt, auslastung_fkt):
    | function autos_neu_fkt = generiere_autos_neu(N_fkt, zeit_abstand_fkt, auslastung_fkt)
    |     zeiten_fkt = zeros(1,N_fkt); %Platzhalter für Spawnzeiten
    |     for i=1:N
    |         zeiten_fkt(i) = zeit_abstand_fkt * i + randn();
    |         if zeiten_fkt(i) < 0
    |             zeiten_fkt(i) = 0
    |         end
    |     end
    | 	
    |     switch (auslastung_fkt)
    |         case 1
    |             wahrscheinlichkeiten = [0.12, 0.20, 0.12, 0.20, 0.12, 0.12, 0.12];
    |         case 2
    |             wahrscheinlichkeiten = [0.08, 0.28, 0.08, 0.28, 0.08, 0.08, 0.12];
    |         case 3
    |             wahrscheinlichkeiten = [0.06, 0.32, 0.085, 0.265, 0.07, 0.12, 0.13];
    |         case 4
    |             wahrscheinlichkeiten = [0.05, 0.2525, 0.14, 0.3175, 0.055, 0.095, 0.14];
    |         case 5
    |             wahrscheinlichkeiten = [0.05, 0.27, 0.135, 0.305, 0.06, 0.095, 0.135];
    |         otherwise
    |             wahrscheinlichkeiten = [0.06, 0.32, 0.07, 0.26, 0.09, 0.12, 0.13];
    |     end
    |     
    |     spuren_werte = [1, 2, 3, 4, 5, 6, 7]; % Die entsprechenden Werte
    | 
    |     kumulative_wahrscheinlichkeiten = cumsum(wahrscheinlichkeiten);
    | 
    |     zufaellige_nummer = rand(1, N_fkt);
    |     spuren = zeros(1, N_fkt); % Platzhalter für die Spuren
    | 
    |     % Werte basierend auf Wahrscheinlichkeiten zuweisen
    |     for i = 1:N_fkt
    |         spuren(i) = spuren_werte(find(zufaellige_nummer(i) <= kumulative_wahrscheinlichkeiten, 1));
    |     end
    | 
    |     zeiten_fkt = sort(zeiten_fkt);
    | 
    |     autos_neu_fkt = [spuren; zeiten_fkt];
    | end
  function [spur1fkt, spur2fkt, spur3fkt, spur4fkt, spur5fkt, spur6fkt, spur7fkt] = spuren_aus_autos(autos_fkt, N_fkt):
    | function [spur1fkt, spur2fkt, spur3fkt, spur4fkt, spur5fkt, spur6fkt, spur7fkt] = spuren_aus_autos(autos_fkt, N_fkt)
    |     counter1 = 1; counter2 = 1; counter3 = 1; counter4 = 1; counter5 = 1; counter6 = 1; counter7 = 1;
    |     spur1fkt = zeros(1,N_fkt/2);
    |     spur2fkt = zeros(1,N_fkt/2);
    |     spur3fkt = zeros(1,N_fkt/2);
    |     spur4fkt = zeros(1,N_fkt/2);
    |     spur5fkt = zeros(1,N_fkt/2);
    |     spur6fkt = zeros(1,N_fkt/2);
    |     spur7fkt = zeros(1,N_fkt/2);
    |     for i = 1:length(autos_fkt)
    |         switch(autos_fkt(1,i))
    |             case 1
    |                 %spur1fkt
    |                 %spur1fkt(counter1)
    |                 %autos_fkt
    |                 %autos_fkt(2,i)
    |                 spur1fkt(counter1) = autos_fkt(2,i);
    |                 counter1 = counter1 + 1;
    |             case 2
    |                 %spur2fkt
    |                 %spur2fkt(counter2)
    |                 %autos_fkt
    |                 %autos_fkt(2,i)
    |                 spur2fkt(counter2) = autos_fkt(2,i);
    |                 counter2 = counter2 + 1;
    |             case 3
    |                 spur3fkt(counter3) = autos_fkt(2,i);
    |                 counter3 = counter3 + 1;
    |             case 4
    |                 spur4fkt(counter4) = autos_fkt(2,i);
    |                 counter4 = counter4 + 1;
    |             case 5
    |                 spur5fkt(counter5) = autos_fkt(2,i);
    |                 counter5 = counter5 + 1;
    |             case 6
    |                 spur6fkt(counter6) = autos_fkt(2,i);
    |                 counter6 = counter6 + 1;
    |             case 7
    |                 spur7fkt(counter7) = autos_fkt(2,i);
